simulink model "model"  (R2014a)
(part 3 of 3)

  bus4 : powerlib/Measurements/Load Flow Bus  LConnTagsString=a  ID=bus4  Vbase=132000  Vref=1  Vangle=0  VLF=1  angleLF=0
      settings: AttributesFormatString=|
      | %<ID>
      | %<Vbase>V
      | %<VLF>pu
      | %<angleLF>deg.
      | %<Name>
  bus40 : powerlib/Measurements/Load Flow Bus  LConnTagsString=a  ID=bus40  Vbase=132000  Vref=1  Vangle=0  VLF=1  angleLF=0
      settings: AttributesFormatString=|
      | %<ID>
      | %<Vbase>V
      | %<VLF>pu
      | %<angleLF>deg.
      | %<Name>
  bus41 : powerlib/Measurements/Load Flow Bus  LConnTagsString=a  ID=bus41  Vbase=132000  Vref=1  Vangle=0  VLF=1  angleLF=0
      settings: AttributesFormatString=|
      | %<ID>
      | %<Vbase>V
      | %<VLF>pu
      | %<angleLF>deg.
      | %<Name>
  bus42 : powerlib/Measurements/Load Flow Bus  LConnTagsString=a  ID=bus42  Vbase=132000  Vref=1  Vangle=0  VLF=1  angleLF=0
      settings: AttributesFormatString=|
      | %<ID>
      | %<Vbase>V
      | %<VLF>pu
      | %<angleLF>deg.
      | %<Name>
  bus43 : powerlib/Measurements/Load Flow Bus  LConnTagsString=a  ID=bus43  Vbase=132000  Vref=1  Vangle=0  VLF=1  angleLF=0
      settings: AttributesFormatString=|
      | %<ID>
      | %<Vbase>V
      | %<VLF>pu
      | %<angleLF>deg.
      | %<Name>
  bus44 : powerlib/Measurements/Load Flow Bus  LConnTagsString=a  ID=bus44  Vbase=132000  Vref=1  Vangle=0  VLF=1  angleLF=0
      settings: AttributesFormatString=|
      | %<ID>
      | %<Vbase>V
      | %<VLF>pu
      | %<angleLF>deg.
      | %<Name>
  bus45 : powerlib/Measurements/Load Flow Bus  LConnTagsString=a  ID=bus45  Vbase=132000  Vref=1  Vangle=0  VLF=1  angleLF=0
      settings: AttributesFormatString=|
      | %<ID>
      | %<Vbase>V
      | %<VLF>pu
      | %<angleLF>deg.
      | %<Name>
  bus46 : powerlib/Measurements/Load Flow Bus  LConnTagsString=a  ID=bus46  Vbase=132000  Vref=1  Vangle=0  VLF=1  angleLF=0
      settings: AttributesFormatString=|
      | %<ID>
      | %<Vbase>V
      | %<VLF>pu
      | %<angleLF>deg.
      | %<Name>
  bus47 : powerlib/Measurements/Load Flow Bus  LConnTagsString=a  ID=bus47  Vbase=132000  Vref=1  Vangle=0  VLF=1  angleLF=0
      settings: AttributesFormatString=|
      | %<ID>
      | %<Vbase>V
      | %<VLF>pu
      | %<angleLF>deg.
      | %<Name>
  bus48 : powerlib/Measurements/Load Flow Bus  LConnTagsString=a  ID=bus48  Vbase=132000  Vref=1  Vangle=0  VLF=1  angleLF=0
      settings: AttributesFormatString=|
      | %<ID>
      | %<Vbase>V
      | %<VLF>pu
      | %<angleLF>deg.
      | %<Name>
  bus49 : powerlib/Measurements/Load Flow Bus  LConnTagsString=a  ID=bus49  Vbase=132000  Vref=1  Vangle=0  VLF=1  angleLF=0
      settings: AttributesFormatString=|
      | %<ID>
      | %<Vbase>V
      | %<VLF>pu
      | %<angleLF>deg.
      | %<Name>
  bus5 : powerlib/Measurements/Load Flow Bus  LConnTagsString=a  ID=bus5  Vbase=132000  Vref=1  Vangle=0  VLF=1  angleLF=0
      settings: AttributesFormatString=|
      | %<ID>
      | %<Vbase>V
      | %<VLF>pu
      | %<angleLF>deg.
      | %<Name>
  bus50 : powerlib/Measurements/Load Flow Bus  LConnTagsString=a  ID=bus50  Vbase=132000  Vref=1  Vangle=0  VLF=1  angleLF=0
      settings: AttributesFormatString=|
      | %<ID>
      | %<Vbase>V
      | %<VLF>pu
      | %<angleLF>deg.
      | %<Name>
  bus51 : powerlib/Measurements/Load Flow Bus  LConnTagsString=a  ID=bus51  Vbase=132000  Vref=1  Vangle=0  VLF=1  angleLF=0
      settings: AttributesFormatString=|
      | %<ID>
      | %<Vbase>V
      | %<VLF>pu
      | %<angleLF>deg.
      | %<Name>
  bus52 : powerlib/Measurements/Load Flow Bus  LConnTagsString=a  ID=bus52  Vbase=132000  Vref=1  Vangle=0  VLF=1  angleLF=0
      settings: AttributesFormatString=|
      | %<ID>
      | %<Vbase>V
      | %<VLF>pu
      | %<angleLF>deg.
      | %<Name>
  bus53 : powerlib/Measurements/Load Flow Bus  LConnTagsString=a  ID=bus53  Vbase=132000  Vref=1  Vangle=0  VLF=1  angleLF=0
      settings: AttributesFormatString=|
      | %<ID>
      | %<Vbase>V
      | %<VLF>pu
      | %<angleLF>deg.
      | %<Name>
  bus54 : powerlib/Measurements/Load Flow Bus  LConnTagsString=a  ID=bus54  Vbase=132000  Vref=1  Vangle=0  VLF=1  angleLF=0
      settings: AttributesFormatString=|
      | %<ID>
      | %<Vbase>V
      | %<VLF>pu
      | %<angleLF>deg.
      | %<Name>
  bus55 : powerlib/Measurements/Load Flow Bus  LConnTagsString=a  ID=bus55  Vbase=132000  Vref=1  Vangle=0  VLF=1  angleLF=0
      settings: AttributesFormatString=|
      | %<ID>
      | %<Vbase>V
      | %<VLF>pu
      | %<angleLF>deg.
      | %<Name>
  bus56 : powerlib/Measurements/Load Flow Bus  LConnTagsString=a  ID=bus56  Vbase=132000  Vref=1  Vangle=0  VLF=1  angleLF=0
      settings: AttributesFormatString=|
      | %<ID>
      | %<Vbase>V
      | %<VLF>pu
      | %<angleLF>deg.
      | %<Name>
  bus57 : powerlib/Measurements/Load Flow Bus  LConnTagsString=a  ID=bus57  Vbase=132000  Vref=1  Vangle=0  VLF=1  angleLF=0
      settings: AttributesFormatString=|
      | %<ID>
      | %<Vbase>V
      | %<VLF>pu
      | %<angleLF>deg.
      | %<Name>
  bus58 : powerlib/Measurements/Load Flow Bus  LConnTagsString=a  ID=bus58  Vbase=132000  Vref=1  Vangle=0  VLF=1  angleLF=0
      settings: AttributesFormatString=|
      | %<ID>
      | %<Vbase>V
      | %<VLF>pu
      | %<angleLF>deg.
      | %<Name>
  bus59 : powerlib/Measurements/Load Flow Bus  LConnTagsString=a  ID=bus59  Vbase=132000  Vref=1  Vangle=0  VLF=1  angleLF=0
      settings: AttributesFormatString=|
      | %<ID>
      | %<Vbase>V
      | %<VLF>pu
      | %<angleLF>deg.
      | %<Name>
  bus6 : powerlib/Measurements/Load Flow Bus  LConnTagsString=a  ID=bus6  Vbase=132000  Vref=1  Vangle=0  VLF=1  angleLF=0
      settings: AttributesFormatString=|
      | %<ID>
      | %<Vbase>V
      | %<VLF>pu
      | %<angleLF>deg.
      | %<Name>
  bus60 : powerlib/Measurements/Load Flow Bus  LConnTagsString=a  ID=bus60  Vbase=132000  Vref=1  Vangle=0  VLF=1  angleLF=0
      settings: AttributesFormatString=|
      | %<ID>
      | %<Vbase>V
      | %<VLF>pu
      | %<angleLF>deg.
      | %<Name>
  bus61 : powerlib/Measurements/Load Flow Bus  LConnTagsString=a  ID=bus61  Vbase=132000  Vref=1  Vangle=0  VLF=1  angleLF=0
      settings: AttributesFormatString=|
      | %<ID>
      | %<Vbase>V
      | %<VLF>pu
      | %<angleLF>deg.
      | %<Name>
  bus62 : powerlib/Measurements/Load Flow Bus  LConnTagsString=a  ID=bus62  Vbase=132000  Vref=1  Vangle=0  VLF=1  angleLF=0
      settings: AttributesFormatString=|
      | %<ID>
      | %<Vbase>V
      | %<VLF>pu
      | %<angleLF>deg.
      | %<Name>
  bus63 : powerlib/Measurements/Load Flow Bus  LConnTagsString=a  ID=bus63  Vbase=132000  Vref=1  Vangle=0  VLF=1  angleLF=0
      settings: AttributesFormatString=|
      | %<ID>
      | %<Vbase>V
      | %<VLF>pu
      | %<angleLF>deg.
      | %<Name>
  bus64 : powerlib/Measurements/Load Flow Bus  LConnTagsString=a  ID=bus64  Vbase=132000  Vref=1  Vangle=0  VLF=1  angleLF=0
      settings: AttributesFormatString=|
      | %<ID>
      | %<Vbase>V
      | %<VLF>pu
      | %<angleLF>deg.
      | %<Name>
  bus65 : powerlib/Measurements/Load Flow Bus  LConnTagsString=a  ID=bus65  Vbase=132000  Vref=1  Vangle=0  VLF=1  angleLF=0
      settings: AttributesFormatString=|
      | %<ID>
      | %<Vbase>V
      | %<VLF>pu
      | %<angleLF>deg.
      | %<Name>
  bus66 : powerlib/Measurements/Load Flow Bus  LConnTagsString=a  ID=bus66  Vbase=132000  Vref=1  Vangle=0  VLF=1  angleLF=0
      settings: AttributesFormatString=|
      | %<ID>
      | %<Vbase>V
      | %<VLF>pu
      | %<angleLF>deg.
      | %<Name>
  bus67 : powerlib/Measurements/Load Flow Bus  LConnTagsString=a  ID=bus67  Vbase=132000  Vref=1  Vangle=0  VLF=1  angleLF=0
      settings: AttributesFormatString=|
      | %<ID>
      | %<Vbase>V
      | %<VLF>pu
      | %<angleLF>deg.
      | %<Name>
  bus68 : powerlib/Measurements/Load Flow Bus  LConnTagsString=a  ID=bus68  Vbase=132000  Vref=1  Vangle=0  VLF=1  angleLF=0
      settings: AttributesFormatString=|
      | %<ID>
      | %<Vbase>V
      | %<VLF>pu
      | %<angleLF>deg.
      | %<Name>
  bus69 : powerlib/Measurements/Load Flow Bus  LConnTagsString=a  ID=bus69  Vbase=132000  Vref=1  Vangle=0  VLF=1  angleLF=0
      settings: AttributesFormatString=|
      | %<ID>
      | %<Vbase>V
      | %<VLF>pu
      | %<angleLF>deg.
      | %<Name>
  bus7 : powerlib/Measurements/Load Flow Bus  LConnTagsString=a  ID=bus7  Vbase=132000  Vref=1  Vangle=0  VLF=1  angleLF=0
      settings: AttributesFormatString=|
      | %<ID>
      | %<Vbase>V
      | %<VLF>pu
      | %<angleLF>deg.
      | %<Name>
  bus70 : powerlib/Measurements/Load Flow Bus  LConnTagsString=a  ID=bus70  Vbase=132000  Vref=1  Vangle=0  VLF=1  angleLF=0
      settings: AttributesFormatString=|
      | %<ID>
      | %<Vbase>V
      | %<VLF>pu
      | %<angleLF>deg.
      | %<Name>
  bus71 : powerlib/Measurements/Load Flow Bus  LConnTagsString=a  ID=bus71  Vbase=132000  Vref=1  Vangle=0  VLF=1  angleLF=0
      settings: AttributesFormatString=|
      | %<ID>
      | %<Vbase>V
      | %<VLF>pu
      | %<angleLF>deg.
      | %<Name>
  bus72 : powerlib/Measurements/Load Flow Bus  LConnTagsString=a  ID=bus72  Vbase=132000  Vref=1  Vangle=0  VLF=1  angleLF=0
      settings: AttributesFormatString=|
      | %<ID>
      | %<Vbase>V
      | %<VLF>pu
      | %<angleLF>deg.
      | %<Name>
  bus73 : powerlib/Measurements/Load Flow Bus  LConnTagsString=a  ID=bus73  Vbase=132000  Vref=1  Vangle=0  VLF=1  angleLF=0
      settings: AttributesFormatString=|
      | %<ID>
      | %<Vbase>V
      | %<VLF>pu
      | %<angleLF>deg.
      | %<Name>
  bus74 : powerlib/Measurements/Load Flow Bus  LConnTagsString=a  ID=bus74  Vbase=132000  Vref=1  Vangle=0  VLF=1  angleLF=0
      settings: AttributesFormatString=|
      | %<ID>
      | %<Vbase>V
      | %<VLF>pu
      | %<angleLF>deg.
      | %<Name>
  bus75 : powerlib/Measurements/Load Flow Bus  LConnTagsString=a  ID=bus75  Vbase=132000  Vref=1  Vangle=0  VLF=1  angleLF=0
      settings: AttributesFormatString=|
      | %<ID>
      | %<Vbase>V
      | %<VLF>pu
      | %<angleLF>deg.
      | %<Name>
  bus76 : powerlib/Measurements/Load Flow Bus  LConnTagsString=a  ID=bus76  Vbase=132000  Vref=1  Vangle=0  VLF=1  angleLF=0
      settings: AttributesFormatString=|
      | %<ID>
      | %<Vbase>V
      | %<VLF>pu
      | %<angleLF>deg.
      | %<Name>
  bus77 : powerlib/Measurements/Load Flow Bus  LConnTagsString=a  ID=bus77  Vbase=132000  Vref=1  Vangle=0  VLF=1  angleLF=0
      settings: AttributesFormatString=|
      | %<ID>
      | %<Vbase>V
      | %<VLF>pu
      | %<angleLF>deg.
      | %<Name>
  bus78 : powerlib/Measurements/Load Flow Bus  LConnTagsString=a  ID=bus78  Vbase=132000  Vref=1  Vangle=0  VLF=1  angleLF=0
      settings: AttributesFormatString=|
      | %<ID>
      | %<Vbase>V
      | %<VLF>pu
      | %<angleLF>deg.
      | %<Name>
  bus79 : powerlib/Measurements/Load Flow Bus  LConnTagsString=a  ID=bus79  Vbase=132000  Vref=1  Vangle=0  VLF=1  angleLF=0
      settings: AttributesFormatString=|
      | %<ID>
      | %<Vbase>V
      | %<VLF>pu
      | %<angleLF>deg.
      | %<Name>
  bus8 : powerlib/Measurements/Load Flow Bus  LConnTagsString=a  ID=bus8  Vbase=132000  Vref=1  Vangle=0  VLF=1  angleLF=0
      settings: AttributesFormatString=|
      | %<ID>
      | %<Vbase>V
      | %<VLF>pu
      | %<angleLF>deg.
      | %<Name>
  bus80 : powerlib/Measurements/Load Flow Bus  LConnTagsString=a  ID=bus80  Vbase=132000  Vref=1  Vangle=0  VLF=1  angleLF=0
      settings: AttributesFormatString=|
      | %<ID>
      | %<Vbase>V
      | %<VLF>pu
      | %<angleLF>deg.
      | %<Name>
  bus81 : powerlib/Measurements/Load Flow Bus  LConnTagsString=a  ID=bus81  Vbase=132000  Vref=1  Vangle=0  VLF=1  angleLF=0
      settings: AttributesFormatString=|
      | %<ID>
      | %<Vbase>V
      | %<VLF>pu
      | %<angleLF>deg.
      | %<Name>
  bus82 : powerlib/Measurements/Load Flow Bus  LConnTagsString=a  ID=bus82  Vbase=132000  Vref=1  Vangle=0  VLF=1  angleLF=0
      settings: AttributesFormatString=|
      | %<ID>
      | %<Vbase>V
      | %<VLF>pu
      | %<angleLF>deg.
      | %<Name>
  bus83 : powerlib/Measurements/Load Flow Bus  LConnTagsString=a  ID=bus83  Vbase=132000  Vref=1  Vangle=0  VLF=1  angleLF=0
      settings: AttributesFormatString=|
      | %<ID>
      | %<Vbase>V
      | %<VLF>pu
      | %<angleLF>deg.
      | %<Name>
  bus84 : powerlib/Measurements/Load Flow Bus  LConnTagsString=a  ID=bus84  Vbase=132000  Vref=1  Vangle=0  VLF=1  angleLF=0
      settings: AttributesFormatString=|
      | %<ID>
      | %<Vbase>V
      | %<VLF>pu
      | %<angleLF>deg.
      | %<Name>
  bus85 : powerlib/Measurements/Load Flow Bus  LConnTagsString=a  ID=bus85  Vbase=132000  Vref=1  Vangle=0  VLF=1  angleLF=0
      settings: AttributesFormatString=|
      | %<ID>
      | %<Vbase>V
      | %<VLF>pu
      | %<angleLF>deg.
      | %<Name>
  bus86 : powerlib/Measurements/Load Flow Bus  LConnTagsString=a  ID=bus86  Vbase=132000  Vref=1  Vangle=0  VLF=1  angleLF=0
      settings: AttributesFormatString=|
      | %<ID>
      | %<Vbase>V
      | %<VLF>pu
      | %<angleLF>deg.
      | %<Name>
  bus87 : powerlib/Measurements/Load Flow Bus  LConnTagsString=a  ID=bus87  Vbase=132000  Vref=1  Vangle=0  VLF=1  angleLF=0
      settings: AttributesFormatString=|
      | %<ID>
      | %<Vbase>V
      | %<VLF>pu
      | %<angleLF>deg.
      | %<Name>
  bus88 : powerlib/Measurements/Load Flow Bus  LConnTagsString=a  ID=bus88  Vbase=132000  Vref=1  Vangle=0  VLF=1  angleLF=0
      settings: AttributesFormatString=|
      | %<ID>
      | %<Vbase>V
      | %<VLF>pu
      | %<angleLF>deg.
      | %<Name>
  bus89 : powerlib/Measurements/Load Flow Bus  LConnTagsString=a  ID=bus89  Vbase=132000  Vref=1  Vangle=0  VLF=1  angleLF=0
      settings: AttributesFormatString=|
      | %<ID>
      | %<Vbase>V
      | %<VLF>pu
      | %<angleLF>deg.
      | %<Name>
  bus9 : powerlib/Measurements/Load Flow Bus  LConnTagsString=a  ID=bus9  Vbase=132000  Vref=1  Vangle=0  VLF=1  angleLF=0
      settings: AttributesFormatString=|
      | %<ID>
      | %<Vbase>V
      | %<VLF>pu
      | %<angleLF>deg.
      | %<Name>
  bus90 : powerlib/Measurements/Load Flow Bus  LConnTagsString=a  ID=bus90  Vbase=132000  Vref=1  Vangle=0  VLF=1  angleLF=0
      settings: AttributesFormatString=|
      | %<ID>
      | %<Vbase>V
      | %<VLF>pu
      | %<angleLF>deg.
      | %<Name>
  bus91 : powerlib/Measurements/Load Flow Bus  LConnTagsString=a  ID=bus91  Vbase=132000  Vref=1  Vangle=0  VLF=1  angleLF=0
      settings: AttributesFormatString=|
      | %<ID>
      | %<Vbase>V
      | %<VLF>pu
      | %<angleLF>deg.
      | %<Name>
  bus92 : powerlib/Measurements/Load Flow Bus  LConnTagsString=a  ID=bus92  Vbase=132000  Vref=1  Vangle=0  VLF=1  angleLF=0
      settings: AttributesFormatString=|
      | %<ID>
      | %<Vbase>V
      | %<VLF>pu
      | %<angleLF>deg.
      | %<Name>
  bus93 : powerlib/Measurements/Load Flow Bus  LConnTagsString=a  ID=bus93  Vbase=132000  Vref=1  Vangle=0  VLF=1  angleLF=0
      settings: AttributesFormatString=|
      | %<ID>
      | %<Vbase>V
      | %<VLF>pu
      | %<angleLF>deg.
      | %<Name>
  bus94 : powerlib/Measurements/Load Flow Bus  LConnTagsString=a  ID=bus94  Vbase=132000  Vref=1  Vangle=0  VLF=1  angleLF=0
      settings: AttributesFormatString=|
      | %<ID>
      | %<Vbase>V
      | %<VLF>pu
      | %<angleLF>deg.
      | %<Name>
  bus95 : powerlib/Measurements/Load Flow Bus  LConnTagsString=a  ID=bus95  Vbase=132000  Vref=1  Vangle=0  VLF=1  angleLF=0
      settings: AttributesFormatString=|
      | %<ID>
      | %<Vbase>V
      | %<VLF>pu
      | %<angleLF>deg.
      | %<Name>
  bus96 : powerlib/Measurements/Load Flow Bus  LConnTagsString=a  ID=bus96  Vbase=132000  Vref=1  Vangle=0  VLF=1  angleLF=0
      settings: AttributesFormatString=|
      | %<ID>
      | %<Vbase>V
      | %<VLF>pu
      | %<angleLF>deg.
      | %<Name>
  bus97 : powerlib/Measurements/Load Flow Bus  LConnTagsString=a  ID=bus97  Vbase=132000  Vref=1  Vangle=0  VLF=1  angleLF=0
      settings: AttributesFormatString=|
      | %<ID>
      | %<Vbase>V
      | %<VLF>pu
      | %<angleLF>deg.
      | %<Name>
  bus98 : powerlib/Measurements/Load Flow Bus  LConnTagsString=a  ID=bus98  Vbase=132000  Vref=1  Vangle=0  VLF=1  angleLF=0
      settings: AttributesFormatString=|
      | %<ID>
      | %<Vbase>V
      | %<VLF>pu
      | %<angleLF>deg.
      | %<Name>
  bus99 : powerlib/Measurements/Load Flow Bus  LConnTagsString=a  ID=bus99  Vbase=132000  Vref=1  Vangle=0  VLF=1  angleLF=0
      settings: AttributesFormatString=|
      | %<ID>
      | %<Vbase>V
      | %<VLF>pu
      | %<angleLF>deg.
      | %<Name>
  powergui : powerlib/powergui  Priority=1  SimulationMode=Continuous  SolverType=Tustin  SampleTime=50e-6  frequency=60  SPID=off  DisableSnubberDevices=off  DisableRonSwitches=off  DisableVfSwitches=off  SwTol=0  Interpol=off  DisplayEquations=off  Ts=0  methode=off  frequencyindice=60  Pbase=100e6  ErrMax=1e-4  Iterations=50  UnitsV=kV  UnitsW=MW  FunctionMessages=off  echomessages=off  HookPort=off  EnableUseOfTLC=off  x0status=blocks  RestoreLinks=warning  ResistiveCurrentMeasurement=off  Frange=[0:2:500]  Ylog=off  Xlog=on  ShowGrid=off  save=off  variable=ZData  structure=0  ZoomFFT=off  StartTime=0.0  cycles=1  DisplayStyle=1  fundamental=60  FreqAxis=off  MaxFrequency=1000  frequencyindicesteady=1  RmsSteady=1  display=off
  connections:
  T_413160960__/LConn1 -- _CN_413160960_132000_CN_413160965_132000/LConn1
  T_413160960__/LConn2 -- _CN_413160960_132000_CN_413160965_132000/LConn2
  _CN_413160960_132000_CN_413160965_132000/LConn3 -- T_413160960__/LConn3 -- bus1/LConn1
  T_413160965__/LConn1 -- _CN_413160960_132000_CN_413160965_132000/RConn1
  T_413160965__/LConn2 -- _CN_413160960_132000_CN_413160965_132000/RConn2
  _CN_413160960_132000_CN_413160965_132000/RConn3 -- T_413160965__/LConn3 -- bus2/LConn1
  T_124680196__/LConn1 -- Puerto_Madryn___Parque_eólico_Loma_Blanca_CN_124680196_132000_CN_429400926_132000/LConn1
  T_124680196__/LConn2 -- Puerto_Madryn___Parque_eólico_Loma_Blanca_CN_124680196_132000_CN_429400926_132000/LConn2
  Puerto_Madryn___Parque_eólico_Loma_Blanca_CN_124680196_132000_CN_429400926_132000/LConn3 -- T_124680196__/LConn3 -- bus3/LConn1
  T_429400926_132000_Estación_Parque_eólico_Loma_Blanca/LConn1 -- Puerto_Madryn___Parque_eólico_Loma_Blanca_CN_124680196_132000_CN_429400926_132000/RConn1
  T_429400926_132000_Estación_Parque_eólico_Loma_Blanca/LConn2 -- Puerto_Madryn___Parque_eólico_Loma_Blanca_CN_124680196_132000_CN_429400926_132000/RConn2
  Puerto_Madryn___Parque_eólico_Loma_Blanca_CN_124680196_132000_CN_429400926_132000/RConn3 -- T_429400926_132000_Estación_Parque_eólico_Loma_Blanca/LConn3 -- bus4/LConn1
  T_313124869__/LConn1 -- _CN_313124869_132000_CN_323007043_132000/LConn1
  T_313124869__/LConn2 -- _CN_313124869_132000_CN_323007043_132000/LConn2
  _CN_313124869_132000_CN_323007043_132000/LConn3 -- T_313124869__/LConn3 -- bus5/LConn1
  _CN_313124869_132000_CN_323007043_132000/RConn1 -- T_323007043__/LConn1 -- _CN_22984932_132000_CN_323007043_132000/LConn1
  _CN_313124869_132000_CN_323007043_132000/RConn2 -- T_323007043__/LConn2 -- _CN_22984932_132000_CN_323007043_132000/LConn2
  _CN_313124869_132000_CN_323007043_132000/RConn3 -- T_323007043__/LConn3 -- _CN_22984932_132000_CN_323007043_132000/LConn3 -- bus6/LConn1
  T_193433094__Estación_transformadora_Santa_Cruz_Norte/LConn1 -- _CN_193433094_132000_CN_299759041_132000/LConn1
  T_193433094__Estación_transformadora_Santa_Cruz_Norte/LConn2 -- _CN_193433094_132000_CN_299759041_132000/LConn2
  _CN_193433094_132000_CN_299759041_132000/LConn3 -- T_193433094__Estación_transformadora_Santa_Cruz_Norte/LConn3 -- bus7/LConn1
  T_299759041__Subestación_transformadora_San_José/LConn1 -- _CN_193433094_132000_CN_299759041_132000/RConn1
  T_299759041__Subestación_transformadora_San_José/LConn2 -- _CN_193433094_132000_CN_299759041_132000/RConn2
  _CN_193433094_132000_CN_299759041_132000/RConn3 -- T_299759041__Subestación_transformadora_San_José/LConn3 -- bus8/LConn1
  T_413160968__/LConn1 -- _CN_413160968_132000_CN_400351708_132000/LConn1
  T_413160968__/LConn2 -- _CN_413160968_132000_CN_400351708_132000/LConn2
  _CN_413160968_132000_CN_400351708_132000/LConn3 -- T_413160968__/LConn3 -- bus9/LConn1
  _CN_413160968_132000_CN_400351708_132000/RConn1 -- T_400351708__Estación_transformadora_Pergamino/LConn1 -- _CN_392660851_132000_CN_400351708_132000/LConn1
  _CN_413160968_132000_CN_400351708_132000/RConn2 -- T_400351708__Estación_transformadora_Pergamino/LConn2 -- _CN_392660851_132000_CN_400351708_132000/LConn2
  _CN_413160968_132000_CN_400351708_132000/RConn3 -- T_400351708__Estación_transformadora_Pergamino/LConn3 -- _CN_392660851_132000_CN_400351708_132000/LConn3 -- bus10/LConn1
  T_413160970__/LConn1 -- _CN_413160970_132000_CN_215284916_132000/LConn1
  T_413160970__/LConn2 -- _CN_413160970_132000_CN_215284916_132000/LConn2
  _CN_413160970_132000_CN_215284916_132000/LConn3 -- T_413160970__/LConn3 -- bus11/LConn1
  _CN_413160970_132000_CN_215284916_132000/RConn1 -- T_215284916_500000_Estación_Transformadora_Campana/LConn1 -- _CN_413160978_132000_CN_215284916_132000/LConn1
  _CN_413160970_132000_CN_215284916_132000/RConn2 -- T_215284916_500000_Estación_Transformadora_Campana/LConn2 -- _CN_413160978_132000_CN_215284916_132000/LConn2
  _CN_413160970_132000_CN_215284916_132000/RConn3 -- T_215284916_500000_Estación_Transformadora_Campana/LConn3 -- _CN_413160978_132000_CN_215284916_132000/LConn3 -- bus12/LConn1
  _CN_321753613_132000_CN_274188832_132000/LConn1 -- T_321753613__/LConn1 -- _CN_321753613_132000_CN_208412024_132000/LConn1
  _CN_321753613_132000_CN_274188832_132000/LConn2 -- T_321753613__/LConn2 -- _CN_321753613_132000_CN_208412024_132000/LConn2
  _CN_321753613_132000_CN_274188832_132000/LConn3 -- T_321753613__/LConn3 -- _CN_321753613_132000_CN_208412024_132000/LConn3 -- bus13/LConn1
  _CN_321753613_132000_CN_274188832_132000/RConn1 -- T_274188832__/LConn1 -- _CN_263644686_132000_CN_274188832_132000/LConn1
  _CN_321753613_132000_CN_274188832_132000/RConn2 -- T_274188832__/LConn2 -- _CN_263644686_132000_CN_274188832_132000/LConn2
  _CN_321753613_132000_CN_274188832_132000/RConn3 -- T_274188832__/LConn3 -- _CN_263644686_132000_CN_274188832_132000/LConn3 -- bus14/LConn1
  _CN_321753613_132000_CN_208412024_132000/RConn1 -- T_208412024__Eléctrica/LConn1 -- _CN_309033575_132000_CN_208412024_132000/LConn1 -- _CN_248861779_132000_CN_208412024_132000/LConn1
  _CN_321753613_132000_CN_208412024_132000/RConn2 -- T_208412024__Eléctrica/LConn2 -- _CN_309033575_132000_CN_208412024_132000/LConn2 -- _CN_248861779_132000_CN_208412024_132000/LConn2
  _CN_321753613_132000_CN_208412024_132000/RConn3 -- T_208412024__Eléctrica/LConn3 -- _CN_309033575_132000_CN_208412024_132000/LConn3 -- bus15/LConn1 -- _CN_248861779_132000_CN_208412024_132000/LConn3
  _CN_263644686_132000_CN_254366935_132000/LConn1 -- T_263644686__/LConn1 -- _CN_263644686_132000_CN_274188832_132000/RConn1
  _CN_263644686_132000_CN_254366935_132000/LConn2 -- T_263644686__/LConn2 -- _CN_263644686_132000_CN_274188832_132000/RConn2
  _CN_263644686_132000_CN_254366935_132000/LConn3 -- T_263644686__/LConn3 -- _CN_263644686_132000_CN_274188832_132000/RConn3 -- bus16/LConn1
  T_254366935__/LConn1 -- _CN_263644686_132000_CN_254366935_132000/RConn1
  T_254366935__/LConn2 -- _CN_263644686_132000_CN_254366935_132000/RConn2
  _CN_263644686_132000_CN_254366935_132000/RConn3 -- T_254366935__/LConn3 -- bus17/LConn1
  T_348404653__/LConn1 -- _CN_348404653_132000_CN_348413858_132000/LConn1
  T_348404653__/LConn2 -- _CN_348404653_132000_CN_348413858_132000/LConn2
  _CN_348404653_132000_CN_348413858_132000/LConn3 -- T_348404653__/LConn3 -- bus18/LConn1
  _CN_348404653_132000_CN_348413858_132000/RConn1 -- T_348413858__/LConn1 -- _CN_255783500_132000_CN_348413858_132000/LConn1 -- _CN_348413858_132000_CN_154839518_132000/LConn1
  _CN_348404653_132000_CN_348413858_132000/RConn2 -- T_348413858__/LConn2 -- _CN_255783500_132000_CN_348413858_132000/LConn2 -- _CN_348413858_132000_CN_154839518_132000/LConn2
  _CN_348404653_132000_CN_348413858_132000/RConn3 -- T_348413858__/LConn3 -- _CN_255783500_132000_CN_348413858_132000/LConn3 -- _CN_348413858_132000_CN_154839518_132000/LConn3 -- bus19/LConn1
  _CN_413160978_132000_CN_413160933_132000/LConn1 -- T_413160978__/LConn1 -- _CN_413160978_132000_CN_215284916_132000/RConn1
  _CN_413160978_132000_CN_413160933_132000/LConn2 -- T_413160978__/LConn2 -- _CN_413160978_132000_CN_215284916_132000/RConn2
  _CN_413160978_132000_CN_413160933_132000/LConn3 -- T_413160978__/LConn3 -- _CN_413160978_132000_CN_215284916_132000/RConn3 -- bus20/LConn1
  T_413160933__/LConn1 -- _CN_413160978_132000_CN_413160933_132000/RConn1
  T_413160933__/LConn2 -- _CN_413160978_132000_CN_413160933_132000/RConn2
  _CN_413160978_132000_CN_413160933_132000/RConn3 -- T_413160933__/LConn3 -- bus21/LConn1
  _CN_314578968_132000_CN_267158870_132000/LConn1 -- T_314578968_132000_/LConn1 -- _CN_314578968_132000_CN_277739296_132000/LConn1 -- _CN_314578968_132000_CN_277641812_132000/LConn1 -- _CN_314578968_132000_CN_276036475_132000/LConn1
  _CN_314578968_132000_CN_267158870_132000/LConn2 -- T_314578968_132000_/LConn2 -- _CN_314578968_132000_CN_277739296_132000/LConn2 -- _CN_314578968_132000_CN_277641812_132000/LConn2 -- _CN_314578968_132000_CN_276036475_132000/LConn2
  _CN_314578968_132000_CN_267158870_132000/LConn3 -- T_314578968_132000_/LConn3 -- _CN_314578968_132000_CN_277739296_132000/LConn3 -- bus22/LConn1 -- _CN_314578968_132000_CN_277641812_132000/LConn3 -- _CN_314578968_132000_CN_276036475_132000/LConn3
  T_267158870__/LConn1 -- _CN_314578968_132000_CN_267158870_132000/RConn1
  T_267158870__/LConn2 -- _CN_314578968_132000_CN_267158870_132000/RConn2
  _CN_314578968_132000_CN_267158870_132000/RConn3 -- T_267158870__/LConn3 -- bus23/LConn1
  _CN_314578968_132000_CN_277641812_132000/RConn1 -- T_277641812__/LConn1 -- _CN_277641812_132000_CN_277641813_132000/LConn1
  _CN_314578968_132000_CN_277641812_132000/RConn2 -- T_277641812__/LConn2 -- _CN_277641812_132000_CN_277641813_132000/LConn2
  _CN_314578968_132000_CN_277641812_132000/RConn3 -- T_277641812__/LConn3 -- _CN_277641812_132000_CN_277641813_132000/LConn3 -- bus24/LConn1
  T_276036475__/LConn1 -- _CN_314578968_132000_CN_276036475_132000/RConn1
  T_276036475__/LConn2 -- _CN_314578968_132000_CN_276036475_132000/RConn2
  _CN_314578968_132000_CN_276036475_132000/RConn3 -- T_276036475__/LConn3 -- bus25/LConn1
  _CN_314578968_132000_CN_277739296_132000/RConn1 -- T_277739296_132000_/LConn1 -- _CN_277739295_132000_CN_277739296_132000/LConn1 -- _CN_277739296_132000_CN_277641813_132000/LConn1 -- _CN_277739296_132000_CN_277739298_132000/LConn1
  _CN_314578968_132000_CN_277739296_132000/RConn2 -- T_277739296_132000_/LConn2 -- _CN_277739295_132000_CN_277739296_132000/LConn2 -- _CN_277739296_132000_CN_277641813_132000/LConn2 -- _CN_277739296_132000_CN_277739298_132000/LConn2
  _CN_314578968_132000_CN_277739296_132000/RConn3 -- T_277739296_132000_/LConn3 -- _CN_277739295_132000_CN_277739296_132000/LConn3 -- _CN_277739296_132000_CN_277641813_132000/LConn3 -- _CN_277739296_132000_CN_277739298_132000/LConn3 -- bus26/LConn1
  _CN_329781274_132000_CN_188145045_132000/LConn1 -- T_329781274__/LConn1 -- _CN_329781274_132000_CN_193707888_132000/LConn1
  _CN_329781274_132000_CN_188145045_132000/LConn2 -- T_329781274__/LConn2 -- _CN_329781274_132000_CN_193707888_132000/LConn2
  _CN_329781274_132000_CN_188145045_132000/LConn3 -- T_329781274__/LConn3 -- _CN_329781274_132000_CN_193707888_132000/LConn3 -- bus27/LConn1
  T_188145045__/LConn1 -- _CN_329781274_132000_CN_188145045_132000/RConn1
  T_188145045__/LConn2 -- _CN_329781274_132000_CN_188145045_132000/RConn2
  _CN_329781274_132000_CN_188145045_132000/RConn3 -- T_188145045__/LConn3 -- bus28/LConn1
  T_193707888__/LConn1 -- _CN_329781274_132000_CN_193707888_132000/RConn1
  T_193707888__/LConn2 -- _CN_329781274_132000_CN_193707888_132000/RConn2
  _CN_329781274_132000_CN_193707888_132000/RConn3 -- T_193707888__/LConn3 -- bus29/LConn1
  _CN_194575899_132000_CN_230950275_132000/LConn1 -- T_194575899__/RConn1 -- _CN_194575899_132000_CN_213353516_132000/LConn1 -- _CN_194575899_132000_CN_214867294_132000/LConn1 -- L_194575899/LConn1
  _CN_194575899_132000_CN_230950275_132000/LConn2 -- T_194575899__/RConn2 -- _CN_194575899_132000_CN_213353516_132000/LConn2 -- _CN_194575899_132000_CN_214867294_132000/LConn2 -- L_194575899/LConn2
  _CN_194575899_132000_CN_230950275_132000/LConn3 -- T_194575899__/RConn3 -- _CN_194575899_132000_CN_213353516_132000/LConn3 -- _CN_194575899_132000_CN_214867294_132000/LConn3 -- L_194575899/LConn3 -- bus30/LConn1
  T_230950275__/LConn1 -- _CN_194575899_132000_CN_230950275_132000/RConn1
  T_230950275__/LConn2 -- _CN_194575899_132000_CN_230950275_132000/RConn2
  _CN_194575899_132000_CN_230950275_132000/RConn3 -- T_230950275__/LConn3 -- bus31/LConn1
  _CN_194575899_132000_CN_213353516_132000/RConn1 -- G_213353516_Central_Nuclear_Embalse/RConn1 -- _CN_213578175_500000_CN_213353516_132000/LConn1 -- _CN_194575899_500000_CN_213353516_132000/LConn1
  _CN_194575899_132000_CN_213353516_132000/RConn2 -- G_213353516_Central_Nuclear_Embalse/RConn2 -- _CN_213578175_500000_CN_213353516_132000/LConn2 -- _CN_194575899_500000_CN_213353516_132000/LConn2
  _CN_194575899_132000_CN_213353516_132000/RConn3 -- G_213353516_Central_Nuclear_Embalse/RConn3 -- _CN_213578175_500000_CN_213353516_132000/LConn3 -- bus32/LConn1 -- _CN_194575899_500000_CN_213353516_132000/LConn3
  T_214867294__/LConn1 -- _CN_194575899_132000_CN_214867294_132000/RConn1
  T_214867294__/LConn2 -- _CN_194575899_132000_CN_214867294_132000/RConn2
  _CN_194575899_132000_CN_214867294_132000/RConn3 -- T_214867294__/LConn3 -- bus33/LConn1
  T_251640352__Subestación_Sudeste/LConn1 -- _CN_251640352_132000_CN_251673647_132000/LConn1
  T_251640352__Subestación_Sudeste/LConn2 -- _CN_251640352_132000_CN_251673647_132000/LConn2
  _CN_251640352_132000_CN_251673647_132000/LConn3 -- T_251640352__Subestación_Sudeste/LConn3 -- bus34/LConn1
  _CN_251640352_132000_CN_251673647_132000/RConn1 -- T_251673647__Subestación_La_Plata/RConn1 -- L_251673647/LConn1
  _CN_251640352_132000_CN_251673647_132000/RConn2 -- T_251673647__Subestación_La_Plata/RConn2 -- L_251673647/LConn2
  _CN_251640352_132000_CN_251673647_132000/RConn3 -- T_251673647__Subestación_La_Plata/RConn3 -- L_251673647/LConn3 -- bus35/LConn1
  T_320719910__/LConn1 -- _CN_320719910_132000_CN_323007038_132000/LConn1
  T_320719910__/LConn2 -- _CN_320719910_132000_CN_323007038_132000/LConn2
  _CN_320719910_132000_CN_323007038_132000/LConn3 -- T_320719910__/LConn3 -- bus36/LConn1
  T_323007038__/LConn1 -- _CN_320719910_132000_CN_323007038_132000/RConn1
  T_323007038__/LConn2 -- _CN_320719910_132000_CN_323007038_132000/RConn2
  _CN_320719910_132000_CN_323007038_132000/RConn3 -- T_323007038__/LConn3 -- bus37/LConn1
  T_381521453__/LConn1 -- _CN_381521453_132000_CN_323007048_132000/LConn1
  T_381521453__/LConn2 -- _CN_381521453_132000_CN_323007048_132000/LConn2
  _CN_381521453_132000_CN_323007048_132000/LConn3 -- T_381521453__/LConn3 -- bus38/LConn1
  _CN_381521453_132000_CN_323007048_132000/RConn1 -- T_323007048__/LConn1 -- _CN_413160959_132000_CN_323007048_132000/LConn1 -- _CN_290602502_132000_CN_323007048_132000/LConn1 -- _CN_323007048_132000_CN_193415212_132000/LConn1
  _CN_381521453_132000_CN_323007048_132000/RConn2 -- T_323007048__/LConn2 -- _CN_413160959_132000_CN_323007048_132000/LConn2 -- _CN_290602502_132000_CN_323007048_132000/LConn2 -- _CN_323007048_132000_CN_193415212_132000/LConn2
  _CN_381521453_132000_CN_323007048_132000/RConn3 -- T_323007048__/LConn3 -- _CN_413160959_132000_CN_323007048_132000/LConn3 -- _CN_290602502_132000_CN_323007048_132000/LConn3 -- _CN_323007048_132000_CN_193415212_132000/LConn3 -- bus39/LConn1
  _CN_199147054_132000_CN_195246048_132000/LConn1 -- T_199147054_132000_Estación_Transformadora_Malvinas/LConn1 -- _CN_199147054_132000_CN_285751980_132000/LConn1
  _CN_199147054_132000_CN_195246048_132000/LConn2 -- T_199147054_132000_Estación_Transformadora_Malvinas/LConn2 -- _CN_199147054_132000_CN_285751980_132000/LConn2
  _CN_199147054_132000_CN_195246048_132000/LConn3 -- T_199147054_132000_Estación_Transformadora_Malvinas/LConn3 -- _CN_199147054_132000_CN_285751980_132000/LConn3 -- bus40/LConn1
  T_195246048__/LConn1 -- _CN_199147054_132000_CN_195246048_132000/RConn1
  T_195246048__/LConn2 -- _CN_199147054_132000_CN_195246048_132000/RConn2
  _CN_199147054_132000_CN_195246048_132000/RConn3 -- T_195246048__/LConn3 -- bus41/LConn1
  T_285751980_132000_Estación_Transformadora_Luján/LConn1 -- _CN_199147054_132000_CN_285751980_132000/RConn1
  T_285751980_132000_Estación_Transformadora_Luján/LConn2 -- _CN_199147054_132000_CN_285751980_132000/RConn2
  _CN_199147054_132000_CN_285751980_132000/RConn3 -- T_285751980_132000_Estación_Transformadora_Luján/LConn3 -- bus42/LConn1
  _CN_323007027_132000_CN_163331032_132000/LConn1 -- T_323007027__/LConn1 -- _CN_323007027_132000_CN_321398723_132000/LConn1
  _CN_323007027_132000_CN_163331032_132000/LConn2 -- T_323007027__/LConn2 -- _CN_323007027_132000_CN_321398723_132000/LConn2
  _CN_323007027_132000_CN_163331032_132000/LConn3 -- T_323007027__/LConn3 -- _CN_323007027_132000_CN_321398723_132000/LConn3 -- bus43/LConn1
  T_163331032__/LConn1 -- _CN_323007027_132000_CN_163331032_132000/RConn1
  T_163331032__/LConn2 -- _CN_323007027_132000_CN_163331032_132000/RConn2
  _CN_323007027_132000_CN_163331032_132000/RConn3 -- T_163331032__/LConn3 -- bus44/LConn1
  _CN_323007027_132000_CN_321398723_132000/RConn1 -- T_321398723__/RConn1 -- _CN_321398723_132000_CN_321398721_132000/LConn1 -- L_321398723/LConn1
  _CN_323007027_132000_CN_321398723_132000/RConn2 -- T_321398723__/RConn2 -- _CN_321398723_132000_CN_321398721_132000/LConn2 -- L_321398723/LConn2
  _CN_323007027_132000_CN_321398723_132000/RConn3 -- T_321398723__/RConn3 -- _CN_321398723_132000_CN_321398721_132000/LConn3 -- L_321398723/LConn3 -- bus45/LConn1
  T_323007032__/LConn1 -- _CN_323007032_132000_CN_323007054_132000/LConn1
  T_323007032__/LConn2 -- _CN_323007032_132000_CN_323007054_132000/LConn2
  _CN_323007032_132000_CN_323007054_132000/LConn3 -- T_323007032__/LConn3 -- bus46/LConn1
  _CN_323007032_132000_CN_323007054_132000/RConn1 -- T_323007054__/LConn1 -- _CN_323007054_132000_CN_272051854_132000/LConn1
  _CN_323007032_132000_CN_323007054_132000/RConn2 -- T_323007054__/LConn2 -- _CN_323007054_132000_CN_272051854_132000/LConn2
  _CN_323007032_132000_CN_323007054_132000/RConn3 -- T_323007054__/LConn3 -- _CN_323007054_132000_CN_272051854_132000/LConn3 -- bus47/LConn1
  T_413160973__/LConn1 -- _CN_413160973_132000_CN_413160958_132000/LConn1
  T_413160973__/LConn2 -- _CN_413160973_132000_CN_413160958_132000/LConn2
  _CN_413160973_132000_CN_413160958_132000/LConn3 -- T_413160973__/LConn3 -- bus48/LConn1
  _CN_413160973_132000_CN_413160958_132000/RConn1 -- T_413160958__/LConn1 -- _CN_290602502_132000_CN_413160958_132000/LConn1
  _CN_413160973_132000_CN_413160958_132000/RConn2 -- T_413160958__/LConn2 -- _CN_290602502_132000_CN_413160958_132000/LConn2
  _CN_413160973_132000_CN_413160958_132000/RConn3 -- T_413160958__/LConn3 -- _CN_290602502_132000_CN_413160958_132000/LConn3 -- bus49/LConn1
  _CN_191859780_132000_CN_323007058_132000/LConn1 -- T_191859780__/RConn1 -- L_191859780/LConn1
  _CN_191859780_132000_CN_323007058_132000/LConn2 -- T_191859780__/RConn2 -- L_191859780/LConn2
  _CN_191859780_132000_CN_323007058_132000/LConn3 -- T_191859780__/RConn3 -- L_191859780/LConn3 -- bus50/LConn1
  _CN_191859780_132000_CN_323007058_132000/RConn1 -- T_323007058__/LConn1 -- _CN_272051854_132000_CN_323007058_132000/LConn1
  _CN_191859780_132000_CN_323007058_132000/RConn2 -- T_323007058__/LConn2 -- _CN_272051854_132000_CN_323007058_132000/LConn2
  _CN_191859780_132000_CN_323007058_132000/RConn3 -- T_323007058__/LConn3 -- _CN_272051854_132000_CN_323007058_132000/LConn3 -- bus51/LConn1
  _CN_58676298_132000_CN_321536940_132000/LConn1 -- T_58676298__Subestación_Edenor/RConn1 -- _CN_58676298_132000_CN_322915916_132000/LConn1 -- L_58676298/LConn1
  _CN_58676298_132000_CN_321536940_132000/LConn2 -- T_58676298__Subestación_Edenor/RConn2 -- _CN_58676298_132000_CN_322915916_132000/LConn2 -- L_58676298/LConn2
  _CN_58676298_132000_CN_321536940_132000/LConn3 -- T_58676298__Subestación_Edenor/RConn3 -- _CN_58676298_132000_CN_322915916_132000/LConn3 -- L_58676298/LConn3 -- bus52/LConn1
  T_321536940__/LConn1 -- _CN_58676298_132000_CN_321536940_132000/RConn1
  T_321536940__/LConn2 -- _CN_58676298_132000_CN_321536940_132000/RConn2
  _CN_58676298_132000_CN_321536940_132000/RConn3 -- T_321536940__/LConn3 -- bus53/LConn1
  T_322915916__/LConn1 -- _CN_58676298_132000_CN_322915916_132000/RConn1
  T_322915916__/LConn2 -- _CN_58676298_132000_CN_322915916_132000/RConn2
  _CN_58676298_132000_CN_322915916_132000/RConn3 -- T_322915916__/LConn3 -- bus54/LConn1
  _CN_255783500_132000_CN_277739294_132000/LConn1 -- T_255783500__/LConn1 -- _CN_255783500_132000_CN_314623617_132000/LConn1 -- _CN_255783500_132000_CN_183904319_132000/LConn1 -- _CN_255783500_132000_CN_348409732_132000/LConn1 -- _CN_255783500_132000_CN_348413858_132000/RConn1
  _CN_255783500_132000_CN_277739294_132000/LConn2 -- T_255783500__/LConn2 -- _CN_255783500_132000_CN_314623617_132000/LConn2 -- _CN_255783500_132000_CN_183904319_132000/LConn2 -- _CN_255783500_132000_CN_348409732_132000/LConn2 -- _CN_255783500_132000_CN_348413858_132000/RConn2
  _CN_255783500_132000_CN_277739294_132000/LConn3 -- T_255783500__/LConn3 -- _CN_255783500_132000_CN_314623617_132000/LConn3 -- _CN_255783500_132000_CN_183904319_132000/LConn3 -- _CN_255783500_132000_CN_348409732_132000/LConn3 -- _CN_255783500_132000_CN_348413858_132000/RConn3 -- bus55/LConn1
  _CN_255783500_132000_CN_277739294_132000/RConn1 -- T_277739294__/LConn1 -- _CN_277739294_132000_CN_277739297_132000/LConn1
  _CN_255783500_132000_CN_277739294_132000/RConn2 -- T_277739294__/LConn2 -- _CN_277739294_132000_CN_277739297_132000/LConn2
  _CN_255783500_132000_CN_277739294_132000/RConn3 -- T_277739294__/LConn3 -- _CN_277739294_132000_CN_277739297_132000/LConn3 -- bus56/LConn1
  T_314623617__/LConn1 -- _CN_255783500_132000_CN_314623617_132000/RConn1
  T_314623617__/LConn2 -- _CN_255783500_132000_CN_314623617_132000/RConn2
  _CN_255783500_132000_CN_314623617_132000/RConn3 -- T_314623617__/LConn3 -- bus57/LConn1
  G_183904319_Central_Termoeléctrica_Necochea/RConn1 -- _CN_255783500_132000_CN_183904319_132000/RConn1
  G_183904319_Central_Termoeléctrica_Necochea/RConn2 -- _CN_255783500_132000_CN_183904319_132000/RConn2
  _CN_255783500_132000_CN_183904319_132000/RConn3 -- G_183904319_Central_Termoeléctrica_Necochea/RConn3 -- bus58/LConn1
  T_348409732__/LConn1 -- _CN_255783500_132000_CN_348409732_132000/RConn1
  T_348409732__/LConn2 -- _CN_255783500_132000_CN_348409732_132000/RConn2
  _CN_255783500_132000_CN_348409732_132000/RConn3 -- T_348409732__/LConn3 -- bus59/LConn1
  _CN_323007054_132000_CN_272051854_132000/RConn1 -- T_272051854__/RConn1 -- _CN_272051854_132000_CN_310571477_132000/LConn1 -- L_272051854/LConn1 -- _CN_272051854_132000_CN_323007058_132000/RConn1
  _CN_323007054_132000_CN_272051854_132000/RConn2 -- T_272051854__/RConn2 -- _CN_272051854_132000_CN_310571477_132000/LConn2 -- L_272051854/LConn2 -- _CN_272051854_132000_CN_323007058_132000/RConn2
  _CN_323007054_132000_CN_272051854_132000/RConn3 -- T_272051854__/RConn3 -- _CN_272051854_132000_CN_310571477_132000/LConn3 -- L_272051854/LConn3 -- bus60/LConn1 -- _CN_272051854_132000_CN_323007058_132000/RConn3
  _CN_193412175_132000_CN_323007050_132000/LConn1 -- T_193412175_500000_Estación_transformadora_Ramallo/RConn4 -- L_193412175/LConn1
  _CN_193412175_132000_CN_323007050_132000/LConn2 -- T_193412175_500000_Estación_transformadora_Ramallo/RConn5 -- L_193412175/LConn2
  _CN_193412175_132000_CN_323007050_132000/LConn3 -- T_193412175_500000_Estación_transformadora_Ramallo/RConn6 -- L_193412175/LConn3 -- bus61/LConn1
  _CN_193412175_132000_CN_323007050_132000/RConn1 -- T_323007050__/LConn1 -- _CN_290602502_132000_CN_323007050_132000/LConn1
  _CN_193412175_132000_CN_323007050_132000/RConn2 -- T_323007050__/LConn2 -- _CN_290602502_132000_CN_323007050_132000/LConn2
  _CN_193412175_132000_CN_323007050_132000/RConn3 -- T_323007050__/LConn3 -- _CN_290602502_132000_CN_323007050_132000/LConn3 -- bus62/LConn1
  T_204494929__Estação_Conversora_de_Frequencia_de_Uruguaiana/LConn1 -- _CN_204494929_132000_CN_204494933_132000/LConn1
  T_204494929__Estação_Conversora_de_Frequencia_de_Uruguaiana/LConn2 -- _CN_204494929_132000_CN_204494933_132000/LConn2
  _CN_204494929_132000_CN_204494933_132000/LConn3 -- T_204494929__Estação_Conversora_de_Frequencia_de_Uruguaiana/LConn3 -- bus63/LConn1
  T_204494933__/LConn1 -- _CN_204494929_132000_CN_204494933_132000/RConn1
  T_204494933__/LConn2 -- _CN_204494929_132000_CN_204494933_132000/RConn2
  _CN_204494929_132000_CN_204494933_132000/RConn3 -- T_204494933__/LConn3 -- bus64/LConn1
  _CN_248861779_132000_CN_208412024_132000/RConn1 -- T_248861779__/LConn1 -- _CN_248861779_132000_CN_323105942_132000/LConn1
  _CN_248861779_132000_CN_208412024_132000/RConn2 -- T_248861779__/LConn2 -- _CN_248861779_132000_CN_323105942_132000/LConn2
  _CN_248861779_132000_CN_208412024_132000/RConn3 -- T_248861779__/LConn3 -- _CN_248861779_132000_CN_323105942_132000/LConn3 -- bus65/LConn1
  _CN_248861779_132000_CN_323105942_132000/RConn1 -- T_323105942__/LConn1 -- _CN_145419356_132000_CN_323105942_132000/LConn1
  _CN_248861779_132000_CN_323105942_132000/RConn2 -- T_323105942__/LConn2 -- _CN_145419356_132000_CN_323105942_132000/LConn2
  _CN_248861779_132000_CN_323105942_132000/RConn3 -- T_323105942__/LConn3 -- _CN_145419356_132000_CN_323105942_132000/LConn3 -- bus66/LConn1
  _CN_277641812_132000_CN_277641813_132000/RConn1 -- T_277641813__/RConn1 -- _CN_432044715_132000_CN_277641813_132000/LConn1 -- _CN_277739296_132000_CN_277641813_132000/RConn1 -- L_277641813/LConn1
  _CN_277641812_132000_CN_277641813_132000/RConn2 -- T_277641813__/RConn2 -- _CN_432044715_132000_CN_277641813_132000/LConn2 -- _CN_277739296_132000_CN_277641813_132000/RConn2 -- L_277641813/LConn2
  _CN_277641812_132000_CN_277641813_132000/RConn3 -- T_277641813__/RConn3 -- _CN_432044715_132000_CN_277641813_132000/LConn3 -- _CN_277739296_132000_CN_277641813_132000/RConn3 -- L_277641813/LConn3 -- bus67/LConn1
  _CN_145419356_132000_CN_422118006_132000/LConn1 -- T_145419356__/LConn1 -- _CN_145419356_132000_CN_130194705_132000/LConn1 -- _CN_145419356_132000_CN_323105942_132000/RConn1
  _CN_145419356_132000_CN_422118006_132000/LConn2 -- T_145419356__/LConn2 -- _CN_145419356_132000_CN_130194705_132000/LConn2 -- _CN_145419356_132000_CN_323105942_132000/RConn2
  _CN_145419356_132000_CN_422118006_132000/LConn3 -- T_145419356__/LConn3 -- _CN_145419356_132000_CN_130194705_132000/LConn3 -- _CN_145419356_132000_CN_323105942_132000/RConn3 -- bus68/LConn1
  T_422118006__/LConn1 -- _CN_145419356_132000_CN_422118006_132000/RConn1
  T_422118006__/LConn2 -- _CN_145419356_132000_CN_422118006_132000/RConn2
  _CN_145419356_132000_CN_422118006_132000/RConn3 -- T_422118006__/LConn3 -- bus69/LConn1
  _CN_145419356_132000_CN_130194705_132000/RConn1 -- T_130194705__/LConn1 -- _CN_130194705_132000_CN_154839518_132000/LConn1
  _CN_145419356_132000_CN_130194705_132000/RConn2 -- T_130194705__/LConn2 -- _CN_130194705_132000_CN_154839518_132000/LConn2
  _CN_145419356_132000_CN_130194705_132000/RConn3 -- T_130194705__/LConn3 -- _CN_130194705_132000_CN_154839518_132000/LConn3 -- bus70/LConn1
  T_284287249__Subestación_Sobral/LConn1 -- _CN_284287249_132000_CN_277938914_132000/LConn1
  T_284287249__Subestación_Sobral/LConn2 -- _CN_284287249_132000_CN_277938914_132000/LConn2
  _CN_284287249_132000_CN_277938914_132000/LConn3 -- T_284287249__Subestación_Sobral/LConn3 -- bus71/LConn1
  T_277938914__/LConn1 -- _CN_284287249_132000_CN_277938914_132000/RConn1
  T_277938914__/LConn2 -- _CN_284287249_132000_CN_277938914_132000/RConn2
  _CN_284287249_132000_CN_277938914_132000/RConn3 -- T_277938914__/LConn3 -- bus72/LConn1
  _CN_309033575_132000_CN_251093639_132000/LConn1 -- T_309033575__/LConn1 -- _CN_309033575_132000_CN_208412024_132000/RConn1
  _CN_309033575_132000_CN_251093639_132000/LConn2 -- T_309033575__/LConn2 -- _CN_309033575_132000_CN_208412024_132000/RConn2
  _CN_309033575_132000_CN_251093639_132000/LConn3 -- T_309033575__/LConn3 -- _CN_309033575_132000_CN_208412024_132000/RConn3 -- bus73/LConn1
  T_251093639_132000_Estación_Transformadora_Verónica/LConn1 -- _CN_309033575_132000_CN_251093639_132000/RConn1
  T_251093639_132000_Estación_Transformadora_Verónica/LConn2 -- _CN_309033575_132000_CN_251093639_132000/RConn2
  _CN_309033575_132000_CN_251093639_132000/RConn3 -- T_251093639_132000_Estación_Transformadora_Verónica/LConn3 -- bus74/LConn1
  _CN_299924594_132000_CN_223678069_132000/LConn1 -- T_299924594__Estación_Pico_Truncado_I/LConn1 -- _CN_299924594_132000_CN_299598854_132000/LConn1
  _CN_299924594_132000_CN_223678069_132000/LConn2 -- T_299924594__Estación_Pico_Truncado_I/LConn2 -- _CN_299924594_132000_CN_299598854_132000/LConn2
  _CN_299924594_132000_CN_223678069_132000/LConn3 -- T_299924594__Estación_Pico_Truncado_I/LConn3 -- _CN_299924594_132000_CN_299598854_132000/LConn3 -- bus75/LConn1
  T_223678069__Estación_transformadora_Puerto_Deseado/LConn1 -- _CN_299924594_132000_CN_223678069_132000/RConn1
  T_223678069__Estación_transformadora_Puerto_Deseado/LConn2 -- _CN_299924594_132000_CN_223678069_132000/RConn2
  _CN_299924594_132000_CN_223678069_132000/RConn3 -- T_223678069__Estación_transformadora_Puerto_Deseado/LConn3 -- bus76/LConn1
  _CN_299924594_132000_CN_299598854_132000/RConn1 -- T_299598854__Estación_transformadora_Las_Heras/LConn1 -- _CN_299598854_132000_CN_317981558_132000/LConn1
  _CN_299924594_132000_CN_299598854_132000/RConn2 -- T_299598854__Estación_transformadora_Las_Heras/LConn2 -- _CN_299598854_132000_CN_317981558_132000/LConn2
  _CN_299924594_132000_CN_299598854_132000/RConn3 -- T_299598854__Estación_transformadora_Las_Heras/LConn3 -- _CN_299598854_132000_CN_317981558_132000/LConn3 -- bus77/LConn1
  T_129988212__Subestación_Transformadora_Transba/LConn1 -- _CN_129988212_132000_CN_257673618_132000/LConn1
  T_129988212__Subestación_Transformadora_Transba/LConn2 -- _CN_129988212_132000_CN_257673618_132000/LConn2
  _CN_129988212_132000_CN_257673618_132000/LConn3 -- T_129988212__Subestación_Transformadora_Transba/LConn3 -- bus78/LConn1
  _CN_129988212_132000_CN_257673618_132000/RConn1 -- T_257673618__/RConn1 -- _CN_257673618_132000_CN_154839518_132000/LConn1 -- L_257673618/LConn1
  _CN_129988212_132000_CN_257673618_132000/RConn2 -- T_257673618__/RConn2 -- _CN_257673618_132000_CN_154839518_132000/LConn2 -- L_257673618/LConn2
  _CN_129988212_132000_CN_257673618_132000/RConn3 -- T_257673618__/RConn3 -- _CN_257673618_132000_CN_154839518_132000/LConn3 -- L_257673618/LConn3 -- bus79/LConn1
  T_322781304__/LConn1 -- _CN_322781304_132000_CN_208425737_132000/LConn1
  T_322781304__/LConn2 -- _CN_322781304_132000_CN_208425737_132000/LConn2
  _CN_322781304_132000_CN_208425737_132000/LConn3 -- T_322781304__/LConn3 -- bus80/LConn1
  _CN_322781304_132000_CN_208425737_132000/RConn1 -- T_208425737__Eléctrica/LConn1 -- _CN_208425737_132000_CN_22984932_132000/LConn1 -- _CN_208425737_132000_CN_431767371_132000/LConn1 -- _CN_208425737_132000_CN_241864152_132000/LConn1
  _CN_322781304_132000_CN_208425737_132000/RConn2 -- T_208425737__Eléctrica/LConn2 -- _CN_208425737_132000_CN_22984932_132000/LConn2 -- _CN_208425737_132000_CN_431767371_132000/LConn2 -- _CN_208425737_132000_CN_241864152_132000/LConn2
  _CN_322781304_132000_CN_208425737_132000/RConn3 -- T_208425737__Eléctrica/LConn3 -- _CN_208425737_132000_CN_22984932_132000/LConn3 -- _CN_208425737_132000_CN_431767371_132000/LConn3 -- _CN_208425737_132000_CN_241864152_132000/LConn3 -- bus81/LConn1
  T_210279051__Estación_Transformadora/LConn1 -- _CN_210279051_132000_CN_283604831_132000/LConn1
  T_210279051__Estación_Transformadora/LConn2 -- _CN_210279051_132000_CN_283604831_132000/LConn2
  _CN_210279051_132000_CN_283604831_132000/LConn3 -- T_210279051__Estación_Transformadora/LConn3 -- bus82/LConn1
  T_283604831__/LConn1 -- _CN_210279051_132000_CN_283604831_132000/RConn1
  T_283604831__/LConn2 -- _CN_210279051_132000_CN_283604831_132000/RConn2
  _CN_210279051_132000_CN_283604831_132000/RConn3 -- T_283604831__/LConn3 -- bus83/LConn1
  _CN_272051854_132000_CN_310571477_132000/RConn1 -- T_310571477__/LConn1 -- _CN_286336657_132000_CN_310571477_132000/LConn1
  _CN_272051854_132000_CN_310571477_132000/RConn2 -- T_310571477__/LConn2 -- _CN_286336657_132000_CN_310571477_132000/LConn2
  _CN_272051854_132000_CN_310571477_132000/RConn3 -- T_310571477__/LConn3 -- _CN_286336657_132000_CN_310571477_132000/LConn3 -- bus84/LConn1
  T_286336657__/LConn1 -- _CN_286336657_132000_CN_310571477_132000/RConn1
  T_286336657__/LConn2 -- _CN_286336657_132000_CN_310571477_132000/RConn2
  _CN_286336657_132000_CN_310571477_132000/RConn3 -- T_286336657__/LConn3 -- bus85/LConn1
  T_413160959__/LConn1 -- _CN_413160959_132000_CN_323007048_132000/RConn1
  T_413160959__/LConn2 -- _CN_413160959_132000_CN_323007048_132000/RConn2
  _CN_413160959_132000_CN_323007048_132000/RConn3 -- T_413160959__/LConn3 -- bus86/LConn1
  T_196031429__/LConn1 -- _CN_196031429_132000_CN_353728814_132000/LConn1
  T_196031429__/LConn2 -- _CN_196031429_132000_CN_353728814_132000/LConn2
  _CN_196031429_132000_CN_353728814_132000/LConn3 -- T_196031429__/LConn3 -- bus87/LConn1
  T_353728814__Estaciòn_Transformadora_San_Miguel/LConn1 -- _CN_196031429_132000_CN_353728814_132000/RConn1
  T_353728814__Estaciòn_Transformadora_San_Miguel/LConn2 -- _CN_196031429_132000_CN_353728814_132000/RConn2
  _CN_196031429_132000_CN_353728814_132000/RConn3 -- T_353728814__Estaciòn_Transformadora_San_Miguel/LConn3 -- bus88/LConn1
  _CN_290602502_132000_CN_413160958_132000/RConn1 -- T_290602502__/LConn1 -- _CN_290602502_132000_CN_323007050_132000/RConn1 -- _CN_290602502_132000_CN_323007048_132000/RConn1
  _CN_290602502_132000_CN_413160958_132000/RConn2 -- T_290602502__/LConn2 -- _CN_290602502_132000_CN_323007050_132000/RConn2 -- _CN_290602502_132000_CN_323007048_132000/RConn2
  _CN_290602502_132000_CN_413160958_132000/RConn3 -- T_290602502__/LConn3 -- _CN_290602502_132000_CN_323007050_132000/RConn3 -- bus89/LConn1 -- _CN_290602502_132000_CN_323007048_132000/RConn3
  _CN_432044715_132000_CN_431976152_132000/LConn1 -- T_432044715__/LConn1 -- _CN_432044715_132000_CN_277641813_132000/RConn1
  _CN_432044715_132000_CN_431976152_132000/LConn2 -- T_432044715__/LConn2 -- _CN_432044715_132000_CN_277641813_132000/RConn2
  _CN_432044715_132000_CN_431976152_132000/LConn3 -- T_432044715__/LConn3 -- _CN_432044715_132000_CN_277641813_132000/RConn3 -- bus90/LConn1
  T_431976152__/LConn1 -- _CN_432044715_132000_CN_431976152_132000/RConn1
  T_431976152__/LConn2 -- _CN_432044715_132000_CN_431976152_132000/RConn2
  _CN_432044715_132000_CN_431976152_132000/RConn3 -- T_431976152__/LConn3 -- bus91/LConn1
  T_306029239__/LConn1 -- _CN_306029239_132000_CN_329781271_132000/LConn1
  T_306029239__/LConn2 -- _CN_306029239_132000_CN_329781271_132000/LConn2
  _CN_306029239_132000_CN_329781271_132000/LConn3 -- T_306029239__/LConn3 -- bus92/LConn1
  T_329781271__/LConn1 -- _CN_306029239_132000_CN_329781271_132000/RConn1
  T_329781271__/LConn2 -- _CN_306029239_132000_CN_329781271_132000/RConn2
  _CN_306029239_132000_CN_329781271_132000/RConn3 -- T_329781271__/LConn3 -- bus93/LConn1
  Trelew___Rawson_CN_429251282_132000_CN_429251283_132000/LConn1 -- T_429251282_132000_Estación_Rawson/LConn1 -- Parque_eólico_Rawson___Rawson_CN_429251282_132000_CN_429251281_132000/LConn1
  Trelew___Rawson_CN_429251282_132000_CN_429251283_132000/LConn2 -- T_429251282_132000_Estación_Rawson/LConn2 -- Parque_eólico_Rawson___Rawson_CN_429251282_132000_CN_429251281_132000/LConn2
  Trelew___Rawson_CN_429251282_132000_CN_429251283_132000/LConn3 -- T_429251282_132000_Estación_Rawson/LConn3 -- Parque_eólico_Rawson___Rawson_CN_429251282_132000_CN_429251281_132000/LConn3 -- bus94/LConn1
  T_429251283_132000_Estación_Trelew/LConn1 -- Trelew___Rawson_CN_429251282_132000_CN_429251283_132000/RConn1
  T_429251283_132000_Estación_Trelew/LConn2 -- Trelew___Rawson_CN_429251282_132000_CN_429251283_132000/RConn2
  Trelew___Rawson_CN_429251282_132000_CN_429251283_132000/RConn3 -- T_429251283_132000_Estación_Trelew/LConn3 -- bus95/LConn1
  T_429251281_132000_Estación_Parque_eólico_Rawson/LConn1 -- Parque_eólico_Rawson___Rawson_CN_429251282_132000_CN_429251281_132000/RConn1
  T_429251281_132000_Estación_Parque_eólico_Rawson/LConn2 -- Parque_eólico_Rawson___Rawson_CN_429251282_132000_CN_429251281_132000/RConn2
  Parque_eólico_Rawson___Rawson_CN_429251282_132000_CN_429251281_132000/RConn3 -- T_429251281_132000_Estación_Parque_eólico_Rawson/LConn3 -- bus96/LConn1
  T_317981558__Subestación_transformadora_Los_Perales_2/LConn1 -- _CN_299598854_132000_CN_317981558_132000/RConn1
  T_317981558__Subestación_transformadora_Los_Perales_2/LConn2 -- _CN_299598854_132000_CN_317981558_132000/RConn2
  _CN_299598854_132000_CN_317981558_132000/RConn3 -- T_317981558__Subestación_transformadora_Los_Perales_2/LConn3 -- bus97/LConn1
  T_277938913__/LConn1 -- _CN_277938913_132000_CN_277938915_132000/LConn1
  T_277938913__/LConn2 -- _CN_277938913_132000_CN_277938915_132000/LConn2
  _CN_277938913_132000_CN_277938915_132000/LConn3 -- T_277938913__/LConn3 -- bus98/LConn1
  T_277938915__/LConn1 -- _CN_277938913_132000_CN_277938915_132000/RConn1
  T_277938915__/LConn2 -- _CN_277938913_132000_CN_277938915_132000/RConn2
  _CN_277938913_132000_CN_277938915_132000/RConn3 -- T_277938915__/LConn3 -- bus99/LConn1
  _CN_203363075_132000_CN_321354632_132000/LConn1 -- T_203363075__/RConn1 -- L_203363075/LConn1
  _CN_203363075_132000_CN_321354632_132000/LConn2 -- T_203363075__/RConn2 -- L_203363075/LConn2
  _CN_203363075_132000_CN_321354632_132000/LConn3 -- T_203363075__/RConn3 -- L_203363075/LConn3 -- bus100/LConn1
  T_321354632__/LConn1 -- _CN_203363075_132000_CN_321354632_132000/RConn1
  T_321354632__/LConn2 -- _CN_203363075_132000_CN_321354632_132000/RConn2
  _CN_203363075_132000_CN_321354632_132000/RConn3 -- T_321354632__/LConn3 -- bus101/LConn1
  _CN_328056071_132000_CN_363050268_132000/LConn1 -- T_328056071__/LConn1 -- _CN_328056071_132000_CN_248651545_132000/LConn1
  _CN_328056071_132000_CN_363050268_132000/LConn2 -- T_328056071__/LConn2 -- _CN_328056071_132000_CN_248651545_132000/LConn2
  _CN_328056071_132000_CN_363050268_132000/LConn3 -- T_328056071__/LConn3 -- _CN_328056071_132000_CN_248651545_132000/LConn3 -- bus102/LConn1
  _CN_328056071_132000_CN_363050268_132000/RConn1 -- T_363050268__Estacion_Transformadora_Villa_Mercedes/LConn1 -- _CN_363050268_132000_CN_211179868_132000/LConn1
  _CN_328056071_132000_CN_363050268_132000/RConn2 -- T_363050268__Estacion_Transformadora_Villa_Mercedes/LConn2 -- _CN_363050268_132000_CN_211179868_132000/LConn2
  _CN_328056071_132000_CN_363050268_132000/RConn3 -- T_363050268__Estacion_Transformadora_Villa_Mercedes/LConn3 -- _CN_363050268_132000_CN_211179868_132000/LConn3 -- bus103/LConn1
  T_248651545__/LConn1 -- _CN_328056071_132000_CN_248651545_132000/RConn1
  T_248651545__/LConn2 -- _CN_328056071_132000_CN_248651545_132000/RConn2
  _CN_328056071_132000_CN_248651545_132000/RConn3 -- T_248651545__/LConn3 -- bus104/LConn1
  _CN_208425737_132000_CN_22984932_132000/RConn1 -- T_22984932__Subestación_de_EDELAP/LConn1 -- _CN_22984932_132000_CN_323007043_132000/RConn1
  _CN_208425737_132000_CN_22984932_132000/RConn2 -- T_22984932__Subestación_de_EDELAP/LConn2 -- _CN_22984932_132000_CN_323007043_132000/RConn2
  _CN_208425737_132000_CN_22984932_132000/RConn3 -- T_22984932__Subestación_de_EDELAP/LConn3 -- _CN_22984932_132000_CN_323007043_132000/RConn3 -- bus105/LConn1
  T_431767371__/LConn1 -- _CN_208425737_132000_CN_431767371_132000/RConn1
  T_431767371__/LConn2 -- _CN_208425737_132000_CN_431767371_132000/RConn2
  _CN_208425737_132000_CN_431767371_132000/RConn3 -- T_431767371__/LConn3 -- bus106/LConn1
  T_241864152__/LConn1 -- _CN_208425737_132000_CN_241864152_132000/RConn1
  T_241864152__/LConn2 -- _CN_208425737_132000_CN_241864152_132000/RConn2
  _CN_208425737_132000_CN_241864152_132000/RConn3 -- T_241864152__/LConn3 -- bus107/LConn1
  _CN_130194705_132000_CN_154839518_132000/RConn1 -- T_154839518__TRANSBA___Subestación_Olavarría___132kV/LConn1 -- _CN_348413858_132000_CN_154839518_132000/RConn1 -- _CN_257673618_132000_CN_154839518_132000/RConn1
  _CN_130194705_132000_CN_154839518_132000/RConn2 -- T_154839518__TRANSBA___Subestación_Olavarría___132kV/LConn2 -- _CN_348413858_132000_CN_154839518_132000/RConn2 -- _CN_257673618_132000_CN_154839518_132000/RConn2
  _CN_130194705_132000_CN_154839518_132000/RConn3 -- T_154839518__TRANSBA___Subestación_Olavarría___132kV/LConn3 -- _CN_348413858_132000_CN_154839518_132000/RConn3 -- bus108/LConn1 -- _CN_257673618_132000_CN_154839518_132000/RConn3
  T_211179868__/LConn1 -- _CN_363050268_132000_CN_211179868_132000/RConn1
  T_211179868__/LConn2 -- _CN_363050268_132000_CN_211179868_132000/RConn2
  _CN_363050268_132000_CN_211179868_132000/RConn3 -- T_211179868__/LConn3 -- bus109/LConn1
  _CN_277739294_132000_CN_277739297_132000/RConn1 -- T_277739297__/LConn1 -- _CN_277739297_132000_CN_277739298_132000/LConn1
  _CN_277739294_132000_CN_277739297_132000/RConn2 -- T_277739297__/LConn2 -- _CN_277739297_132000_CN_277739298_132000/LConn2
  _CN_277739294_132000_CN_277739297_132000/RConn3 -- T_277739297__/LConn3 -- _CN_277739297_132000_CN_277739298_132000/LConn3 -- bus110/LConn1
  T_277739295_132000_/LConn1 -- _CN_277739295_132000_CN_277739296_132000/RConn1
  T_277739295_132000_/LConn2 -- _CN_277739295_132000_CN_277739296_132000/RConn2
  _CN_277739295_132000_CN_277739296_132000/RConn3 -- T_277739295_132000_/LConn3 -- bus111/LConn1
  _CN_277739296_132000_CN_277739298_132000/RConn1 -- T_277739298__/LConn1 -- _CN_277739297_132000_CN_277739298_132000/RConn1
  _CN_277739296_132000_CN_277739298_132000/RConn2 -- T_277739298__/LConn2 -- _CN_277739297_132000_CN_277739298_132000/RConn2
  _CN_277739296_132000_CN_277739298_132000/RConn3 -- T_277739298__/LConn3 -- _CN_277739297_132000_CN_277739298_132000/RConn3 -- bus112/LConn1
  _CN_179545958_132000_CN_321354631_132000/LConn1 -- T_179545958_500000_Estación_Transformadora_Ezeiza/RConn4 -- L_179545958/LConn1
  _CN_179545958_132000_CN_321354631_132000/LConn2 -- T_179545958_500000_Estación_Transformadora_Ezeiza/RConn5 -- L_179545958/LConn2
  _CN_179545958_132000_CN_321354631_132000/LConn3 -- T_179545958_500000_Estación_Transformadora_Ezeiza/RConn6 -- L_179545958/LConn3 -- bus113/LConn1
  T_321354631__/LConn1 -- _CN_179545958_132000_CN_321354631_132000/RConn1
  T_321354631__/LConn2 -- _CN_179545958_132000_CN_321354631_132000/RConn2
  _CN_179545958_132000_CN_321354631_132000/RConn3 -- T_321354631__/LConn3 -- bus114/LConn1
  T_340060050_500000_Estación_Transformadora_Centro/LConn1 -- _CN_340060050_132000_CN_97399680_132000/LConn1
  T_340060050_500000_Estación_Transformadora_Centro/LConn2 -- _CN_340060050_132000_CN_97399680_132000/LConn2
  _CN_340060050_132000_CN_97399680_132000/LConn3 -- T_340060050_500000_Estación_Transformadora_Centro/LConn3 -- bus115/LConn1
  T_97399680_500000_Estación_Transformadora_San_Isidro/LConn1 -- _CN_340060050_132000_CN_97399680_132000/RConn1
  T_97399680_500000_Estación_Transformadora_San_Isidro/LConn2 -- _CN_340060050_132000_CN_97399680_132000/RConn2
  _CN_340060050_132000_CN_97399680_132000/RConn3 -- T_97399680_500000_Estación_Transformadora_San_Isidro/LConn3 -- bus116/LConn1
  T_392660851__/LConn1 -- _CN_392660851_132000_CN_400351708_132000/RConn1
  T_392660851__/LConn2 -- _CN_392660851_132000_CN_400351708_132000/RConn2
  _CN_392660851_132000_CN_400351708_132000/RConn3 -- T_392660851__/LConn3 -- bus117/LConn1
  T_326097046__/LConn1 -- _CN_326097046_132000_CN_314176103_132000/LConn1
  T_326097046__/LConn2 -- _CN_326097046_132000_CN_314176103_132000/LConn2
  _CN_326097046_132000_CN_314176103_132000/LConn3 -- T_326097046__/LConn3 -- bus118/LConn1
  _CN_326097046_132000_CN_314176103_132000/RConn1 -- T_314176103__Estación_transformadora_Esperanza/RConn1 -- L_314176103/LConn1
  _CN_326097046_132000_CN_314176103_132000/RConn2 -- T_314176103__Estación_transformadora_Esperanza/RConn2 -- L_314176103/LConn2
  _CN_326097046_132000_CN_314176103_132000/RConn3 -- T_314176103__Estación_transformadora_Esperanza/RConn3 -- L_314176103/LConn3 -- bus119/LConn1
  T_230329765__/LConn1 -- _CN_230329765_132000_CN_322781303_132000/LConn1
  T_230329765__/LConn2 -- _CN_230329765_132000_CN_322781303_132000/LConn2
  _CN_230329765_132000_CN_322781303_132000/LConn3 -- T_230329765__/LConn3 -- bus120/LConn1
  T_322781303__/LConn1 -- _CN_230329765_132000_CN_322781303_132000/RConn1
  T_322781303__/LConn2 -- _CN_230329765_132000_CN_322781303_132000/RConn2
  _CN_230329765_132000_CN_322781303_132000/RConn3 -- T_322781303__/LConn3 -- bus121/LConn1
  _CN_323007048_132000_CN_193415212_132000/RConn1 -- G_193415212_Central_Nuclear_de_Atucha_I/RConn1 -- 2ATVL1Y2_CN_277132135_220000_CN_193415212_132000/LConn1 -- _CN_193412175_500000_CN_193415212_132000/LConn1 -- _CN_199287768_500000_CN_193415212_132000/LConn1
  _CN_323007048_132000_CN_193415212_132000/RConn2 -- G_193415212_Central_Nuclear_de_Atucha_I/RConn2 -- 2ATVL1Y2_CN_277132135_220000_CN_193415212_132000/LConn2 -- _CN_193412175_500000_CN_193415212_132000/LConn2 -- _CN_199287768_500000_CN_193415212_132000/LConn2
  _CN_323007048_132000_CN_193415212_132000/RConn3 -- G_193415212_Central_Nuclear_de_Atucha_I/RConn3 -- 2ATVL1Y2_CN_277132135_220000_CN_193415212_132000/LConn3 -- _CN_193412175_500000_CN_193415212_132000/LConn3 -- _CN_199287768_500000_CN_193415212_132000/LConn3 -- bus122/LConn1
  T_321398721__/LConn1 -- _CN_321398723_132000_CN_321398721_132000/RConn1
  T_321398721__/LConn2 -- _CN_321398723_132000_CN_321398721_132000/RConn2
  _CN_321398723_132000_CN_321398721_132000/RConn3 -- T_321398721__/LConn3 -- bus123/LConn1
  T_259688907__/LConn1 -- _CN_259688907_132000_CN_230070479_132000/LConn1
  T_259688907__/LConn2 -- _CN_259688907_132000_CN_230070479_132000/LConn2
  _CN_259688907_132000_CN_230070479_132000/LConn3 -- T_259688907__/LConn3 -- bus124/LConn1
  G_230070479_Planta_Generadora_C_L_Y_F_E_M_A_/RConn1 -- _CN_259688907_132000_CN_230070479_132000/RConn1
  G_230070479_Planta_Generadora_C_L_Y_F_E_M_A_/RConn2 -- _CN_259688907_132000_CN_230070479_132000/RConn2
  _CN_259688907_132000_CN_230070479_132000/RConn3 -- G_230070479_Planta_Generadora_C_L_Y_F_E_M_A_/RConn3 -- bus125/LConn1
  _CN_203363075_220000_CN_179545958_220000/LConn1 -- T_203363075__/LConn1 -- _CN_203363075_220000_CN_431598950_220000/LConn1
  _CN_203363075_220000_CN_179545958_220000/LConn2 -- T_203363075__/LConn2 -- _CN_203363075_220000_CN_431598950_220000/LConn2
  _CN_203363075_220000_CN_179545958_220000/LConn3 -- T_203363075__/LConn3 -- _CN_203363075_220000_CN_431598950_220000/LConn3 -- bus126/LConn1
  _CN_203363075_220000_CN_179545958_220000/RConn1 -- T_179545958_500000_Estación_Transformadora_Ezeiza/RConn1 -- _CN_172440613_220000_CN_179545958_220000/LConn1 -- _CN_321398723_220000_CN_179545958_220000/LConn1 -- _CN_58676298_220000_CN_179545958_220000/LConn1
  _CN_203363075_220000_CN_179545958_220000/RConn2 -- T_179545958_500000_Estación_Transformadora_Ezeiza/RConn2 -- _CN_172440613_220000_CN_179545958_220000/LConn2 -- _CN_321398723_220000_CN_179545958_220000/LConn2 -- _CN_58676298_220000_CN_179545958_220000/LConn2
  _CN_203363075_220000_CN_179545958_220000/RConn3 -- T_179545958_500000_Estación_Transformadora_Ezeiza/RConn3 -- _CN_172440613_220000_CN_179545958_220000/LConn3 -- _CN_321398723_220000_CN_179545958_220000/LConn3 -- _CN_58676298_220000_CN_179545958_220000/LConn3 -- bus127/LConn1
  _CN_203363075_220000_CN_431598950_220000/RConn1 -- T_431598950__/LConn1 -- _CN_242365381_220000_CN_431598950_220000/LConn1
  _CN_203363075_220000_CN_431598950_220000/RConn2 -- T_431598950__/LConn2 -- _CN_242365381_220000_CN_431598950_220000/LConn2
  _CN_203363075_220000_CN_431598950_220000/RConn3 -- T_431598950__/LConn3 -- _CN_242365381_220000_CN_431598950_220000/LConn3 -- bus128/LConn1
  T_164577670__Estación_Electrica/LConn1 -- _CN_164577670_220000_CN_164673290_220000/LConn1
  T_164577670__Estación_Electrica/LConn2 -- _CN_164577670_220000_CN_164673290_220000/LConn2
  _CN_164577670_220000_CN_164673290_220000/LConn3 -- T_164577670__Estación_Electrica/LConn3 -- bus129/LConn1
  T_164673290__/LConn1 -- _CN_164577670_220000_CN_164673290_220000/RConn1
  T_164673290__/LConn2 -- _CN_164577670_220000_CN_164673290_220000/RConn2
  _CN_164577670_220000_CN_164673290_220000/RConn3 -- T_164673290__/LConn3 -- bus130/LConn1
  T_272051854__/LConn1 -- _CN_272051854_220000_CN_199287768_220000/LConn1
  T_272051854__/LConn2 -- _CN_272051854_220000_CN_199287768_220000/LConn2
  _CN_272051854_220000_CN_199287768_220000/LConn3 -- T_272051854__/LConn3 -- bus131/LConn1
  _CN_272051854_220000_CN_199287768_220000/RConn1 -- T_199287768_500000_Estación_Transformadora_General_Rodríguez/RConn1 -- _CN_199287768_220000_CN_277132135_220000/LConn1 -- L_199287768/LConn1 -- _CN_191859780_220000_CN_199287768_220000/LConn1
  _CN_272051854_220000_CN_199287768_220000/RConn2 -- T_199287768_500000_Estación_Transformadora_General_Rodríguez/RConn2 -- _CN_199287768_220000_CN_277132135_220000/LConn2 -- L_199287768/LConn2 -- _CN_191859780_220000_CN_199287768_220000/LConn2
  _CN_272051854_220000_CN_199287768_220000/RConn3 -- T_199287768_500000_Estación_Transformadora_General_Rodríguez/RConn3 -- _CN_199287768_220000_CN_277132135_220000/LConn3 -- L_199287768/LConn3 -- bus132/LConn1 -- _CN_191859780_220000_CN_199287768_220000/LConn3
  T_251673647__Subestación_La_Plata/LConn1 -- _CN_251673647_220000_CN_251081502_220000/LConn1
  T_251673647__Subestación_La_Plata/LConn2 -- _CN_251673647_220000_CN_251081502_220000/LConn2
  _CN_251673647_220000_CN_251081502_220000/LConn3 -- T_251673647__Subestación_La_Plata/LConn3 -- bus133/LConn1
  _CN_251673647_220000_CN_251081502_220000/RConn1 -- T_251081502_220000;500000_Estación_Transformadora_Abasto/RConn1 -- L_251081502/LConn1
  _CN_251673647_220000_CN_251081502_220000/RConn2 -- T_251081502_220000;500000_Estación_Transformadora_Abasto/RConn2 -- L_251081502/LConn2
  _CN_251673647_220000_CN_251081502_220000/RConn3 -- T_251081502_220000;500000_Estación_Transformadora_Abasto/RConn3 -- L_251081502/LConn3 -- bus134/LConn1
  T_273522974__/LConn1 -- _CN_273522974_220000_CN_285554517_220000/LConn1
  T_273522974__/LConn2 -- _CN_273522974_220000_CN_285554517_220000/LConn2
  _CN_273522974_220000_CN_285554517_220000/LConn3 -- T_273522974__/LConn3 -- bus135/LConn1
  _CN_273522974_220000_CN_285554517_220000/RConn1 -- T_285554517__/LConn1 -- _CN_285554517_220000_CN_285554522_220000/LConn1
  _CN_273522974_220000_CN_285554517_220000/RConn2 -- T_285554517__/LConn2 -- _CN_285554517_220000_CN_285554522_220000/LConn2
  _CN_273522974_220000_CN_285554517_220000/RConn3 -- T_285554517__/LConn3 -- _CN_285554517_220000_CN_285554522_220000/LConn3 -- bus136/LConn1
  T_172440613__/LConn1 -- _CN_172440613_220000_CN_179545958_220000/RConn1
  T_172440613__/LConn2 -- _CN_172440613_220000_CN_179545958_220000/RConn2
  _CN_172440613_220000_CN_179545958_220000/RConn3 -- T_172440613__/LConn3 -- bus137/LConn1
  _CN_193242927_220000_CN_191859780_220000/LConn1 -- T_193242927__/LConn1 -- _CN_193242927_220000_CN_178248568_220000/LConn1
  _CN_193242927_220000_CN_191859780_220000/LConn2 -- T_193242927__/LConn2 -- _CN_193242927_220000_CN_178248568_220000/LConn2
  _CN_193242927_220000_CN_191859780_220000/LConn3 -- T_193242927__/LConn3 -- _CN_193242927_220000_CN_178248568_220000/LConn3 -- bus138/LConn1
  _CN_193242927_220000_CN_191859780_220000/RConn1 -- T_191859780__/LConn1 -- _CN_191859780_220000_CN_199287768_220000/RConn1
  _CN_193242927_220000_CN_191859780_220000/RConn2 -- T_191859780__/LConn2 -- _CN_191859780_220000_CN_199287768_220000/RConn2
  _CN_193242927_220000_CN_191859780_220000/RConn3 -- T_191859780__/LConn3 -- _CN_191859780_220000_CN_199287768_220000/RConn3 -- bus139/LConn1
  _CN_193242927_220000_CN_178248568_220000/RConn1 -- T_178248568__/LConn1 -- _CN_310114524_220000_CN_178248568_220000/LConn1
  _CN_193242927_220000_CN_178248568_220000/RConn2 -- T_178248568__/LConn2 -- _CN_310114524_220000_CN_178248568_220000/LConn2
  _CN_193242927_220000_CN_178248568_220000/RConn3 -- T_178248568__/LConn3 -- _CN_310114524_220000_CN_178248568_220000/LConn3 -- bus140/LConn1
  T_321398723__/LConn1 -- _CN_321398723_220000_CN_179545958_220000/RConn1
  T_321398723__/LConn2 -- _CN_321398723_220000_CN_179545958_220000/RConn2
  _CN_321398723_220000_CN_179545958_220000/RConn3 -- T_321398723__/LConn3 -- bus141/LConn1
  T_242365381__/LConn1 -- _CN_242365381_220000_CN_431598950_220000/RConn1
  T_242365381__/LConn2 -- _CN_242365381_220000_CN_431598950_220000/RConn2
  _CN_242365381_220000_CN_431598950_220000/RConn3 -- T_242365381__/LConn3 -- bus142/LConn1
  T_58676298__Subestación_Edenor/LConn1 -- _CN_58676298_220000_CN_179545958_220000/RConn1
  T_58676298__Subestación_Edenor/LConn2 -- _CN_58676298_220000_CN_179545958_220000/RConn2
  _CN_58676298_220000_CN_179545958_220000/RConn3 -- T_58676298__Subestación_Edenor/LConn3 -- bus143/LConn1
  2RAVL1Y2_CN_193412175_220000_CN_277132135_220000/LConn1 -- T_193412175_500000_Estación_transformadora_Ramallo/RConn1 -- _CN_193412175_220000_CN_194378395_220000/LConn1
  2RAVL1Y2_CN_193412175_220000_CN_277132135_220000/LConn2 -- T_193412175_500000_Estación_transformadora_Ramallo/RConn2 -- _CN_193412175_220000_CN_194378395_220000/LConn2
  2RAVL1Y2_CN_193412175_220000_CN_277132135_220000/LConn3 -- T_193412175_500000_Estación_transformadora_Ramallo/RConn3 -- _CN_193412175_220000_CN_194378395_220000/LConn3 -- bus144/LConn1
  2RAVL1Y2_CN_193412175_220000_CN_277132135_220000/RConn1 -- T_277132135_220000_Estación_transformadora_Villa_Lía/LConn1 -- _CN_199287768_220000_CN_277132135_220000/RConn1 -- 2ATVL1Y2_CN_277132135_220000_CN_193415212_132000/RConn1
  2RAVL1Y2_CN_193412175_220000_CN_277132135_220000/RConn2 -- T_277132135_220000_Estación_transformadora_Villa_Lía/LConn2 -- _CN_199287768_220000_CN_277132135_220000/RConn2 -- 2ATVL1Y2_CN_277132135_220000_CN_193415212_132000/RConn2
  2RAVL1Y2_CN_193412175_220000_CN_277132135_220000/RConn3 -- T_277132135_220000_Estación_transformadora_Villa_Lía/LConn3 -- _CN_199287768_220000_CN_277132135_220000/RConn3 -- 2ATVL1Y2_CN_277132135_220000_CN_193415212_132000/RConn3 -- bus145/LConn1
  G_194378395_Argener/RConn1 -- _CN_193412175_220000_CN_194378395_220000/RConn1
  G_194378395_Argener/RConn2 -- _CN_193412175_220000_CN_194378395_220000/RConn2
  _CN_193412175_220000_CN_194378395_220000/RConn3 -- G_194378395_Argener/RConn3 -- bus146/LConn1
  G_285554522_Central_Eléctrica_Barragán/RConn1 -- _CN_285554517_220000_CN_285554522_220000/RConn1
  G_285554522_Central_Eléctrica_Barragán/RConn2 -- _CN_285554517_220000_CN_285554522_220000/RConn2
  _CN_285554517_220000_CN_285554522_220000/RConn3 -- G_285554522_Central_Eléctrica_Barragán/RConn3 -- bus147/LConn1
  T_310114524__Subestación_Edenor/LConn1 -- _CN_310114524_220000_CN_178248568_220000/RConn1
  T_310114524__Subestación_Edenor/LConn2 -- _CN_310114524_220000_CN_178248568_220000/RConn2
  _CN_310114524_220000_CN_178248568_220000/RConn3 -- T_310114524__Subestación_Edenor/LConn3 -- bus148/LConn1
  _CN_188360578_500000_CN_247830316_500000/LConn1 -- T_188360578__/LConn1 -- _CN_188360578_500000_CN_413038969_500000/LConn1
  _CN_188360578_500000_CN_247830316_500000/LConn2 -- T_188360578__/LConn2 -- _CN_188360578_500000_CN_413038969_500000/LConn2
  _CN_188360578_500000_CN_247830316_500000/LConn3 -- T_188360578__/LConn3 -- _CN_188360578_500000_CN_413038969_500000/LConn3 -- bus149/LConn1
  _CN_188360578_500000_CN_247830316_500000/RConn1 -- T_247830316__/LConn1 -- _CN_247830316_500000_CN_218457595_500000/LConn1 -- _CN_247830316_500000_CN_176046623_500000/LConn1
  _CN_188360578_500000_CN_247830316_500000/RConn2 -- T_247830316__/LConn2 -- _CN_247830316_500000_CN_218457595_500000/LConn2 -- _CN_247830316_500000_CN_176046623_500000/LConn2
  _CN_188360578_500000_CN_247830316_500000/RConn3 -- T_247830316__/LConn3 -- _CN_247830316_500000_CN_218457595_500000/LConn3 -- bus150/LConn1 -- _CN_247830316_500000_CN_176046623_500000/LConn3
  _CN_188360578_500000_CN_413038969_500000/RConn1 -- T_413038969__/LConn1 -- _CN_26119134_500000_CN_413038969_500000/LConn1 -- _CN_413038969_500000_CN_178480305_500000/LConn1 -- _CN_213192904_500000_CN_413038969_500000/LConn1
  _CN_188360578_500000_CN_413038969_500000/RConn2 -- T_413038969__/LConn2 -- _CN_26119134_500000_CN_413038969_500000/LConn2 -- _CN_413038969_500000_CN_178480305_500000/LConn2 -- _CN_213192904_500000_CN_413038969_500000/LConn2
  _CN_188360578_500000_CN_413038969_500000/RConn3 -- T_413038969__/LConn3 -- _CN_26119134_500000_CN_413038969_500000/LConn3 -- _CN_413038969_500000_CN_178480305_500000/LConn3 -- bus151/LConn1 -- _CN_213192904_500000_CN_413038969_500000/LConn3
  _CN_277426564_500000_CN_277641813_500000/LConn1 -- T_277426564__/LConn1 -- _CN_277426564_500000_CN_251081502_500000/LConn1
  _CN_277426564_500000_CN_277641813_500000/LConn2 -- T_277426564__/LConn2 -- _CN_277426564_500000_CN_251081502_500000/LConn2
  _CN_277426564_500000_CN_277641813_500000/LConn3 -- T_277426564__/LConn3 -- _CN_277426564_500000_CN_251081502_500000/LConn3 -- bus152/LConn1
  _CN_277426564_500000_CN_277641813_500000/RConn1 -- T_277641813__/LConn1 -- _CN_71775909_500000_CN_277641813_500000/LConn1 -- _CN_277641813_500000_CN_26119134_500000/LConn1
  _CN_277426564_500000_CN_277641813_500000/RConn2 -- T_277641813__/LConn2 -- _CN_71775909_500000_CN_277641813_500000/LConn2 -- _CN_277641813_500000_CN_26119134_500000/LConn2
  _CN_277426564_500000_CN_277641813_500000/RConn3 -- T_277641813__/LConn3 -- _CN_71775909_500000_CN_277641813_500000/LConn3 -- _CN_277641813_500000_CN_26119134_500000/LConn3 -- bus153/LConn1
  _CN_277426564_500000_CN_251081502_500000/RConn1 -- T_251081502_220000;500000_Estación_Transformadora_Abasto/LConn1 -- _CN_251081502_500000_CN_179545958_500000/LConn1
  _CN_277426564_500000_CN_251081502_500000/RConn2 -- T_251081502_220000;500000_Estación_Transformadora_Abasto/LConn2 -- _CN_251081502_500000_CN_179545958_500000/LConn2
  _CN_277426564_500000_CN_251081502_500000/RConn3 -- T_251081502_220000;500000_Estación_Transformadora_Abasto/LConn3 -- _CN_251081502_500000_CN_179545958_500000/LConn3 -- bus154/LConn1
  _CN_247830316_500000_CN_176046623_500000/RConn1 -- T_176046623__/LConn1 -- _CN_176046623_500000_CN_247830317_500000/LConn1
  _CN_247830316_500000_CN_176046623_500000/RConn2 -- T_176046623__/LConn2 -- _CN_176046623_500000_CN_247830317_500000/LConn2
  _CN_247830316_500000_CN_176046623_500000/RConn3 -- T_176046623__/LConn3 -- _CN_176046623_500000_CN_247830317_500000/LConn3 -- bus155/LConn1
  T_218457595__/LConn1 -- _CN_247830316_500000_CN_218457595_500000/RConn1
  T_218457595__/LConn2 -- _CN_247830316_500000_CN_218457595_500000/RConn2
  _CN_247830316_500000_CN_218457595_500000/RConn3 -- T_218457595__/LConn3 -- bus156/LConn1
  _CN_110339851_500000_CN_258696364_500000/LConn1 -- T_110339851__Estación_Transformadora_Puerto_Bastiani/LConn1 -- _CN_110339851_500000_CN_305162903_500000/LConn1 -- _CN_110339851_500000_CN_258696366_500000/LConn1
  _CN_110339851_500000_CN_258696364_500000/LConn2 -- T_110339851__Estación_Transformadora_Puerto_Bastiani/LConn2 -- _CN_110339851_500000_CN_305162903_500000/LConn2 -- _CN_110339851_500000_CN_258696366_500000/LConn2
  _CN_110339851_500000_CN_258696364_500000/LConn3 -- T_110339851__Estación_Transformadora_Puerto_Bastiani/LConn3 -- _CN_110339851_500000_CN_305162903_500000/LConn3 -- bus157/LConn1 -- _CN_110339851_500000_CN_258696366_500000/LConn3
  _CN_110339851_500000_CN_258696364_500000/RConn1 -- T_258696364__/LConn1 -- _CN_258696364_500000_CN_221357412_500000/LConn1
  _CN_110339851_500000_CN_258696364_500000/RConn2 -- T_258696364__/LConn2 -- _CN_258696364_500000_CN_221357412_500000/LConn2
  _CN_110339851_500000_CN_258696364_500000/RConn3 -- T_258696364__/LConn3 -- _CN_258696364_500000_CN_221357412_500000/LConn3 -- bus158/LConn1
  _CN_110339851_500000_CN_258696366_500000/RConn1 -- T_258696366__/LConn1 -- _CN_305027751_500000_CN_258696366_500000/LConn1
  _CN_110339851_500000_CN_258696366_500000/RConn2 -- T_258696366__/LConn2 -- _CN_305027751_500000_CN_258696366_500000/LConn2
  _CN_110339851_500000_CN_258696366_500000/RConn3 -- T_258696366__/LConn3 -- _CN_305027751_500000_CN_258696366_500000/LConn3 -- bus159/LConn1
  T_305162903__/LConn1 -- _CN_110339851_500000_CN_305162903_500000/RConn1
  T_305162903__/LConn2 -- _CN_110339851_500000_CN_305162903_500000/RConn2
  _CN_110339851_500000_CN_305162903_500000/RConn3 -- T_305162903__/LConn3 -- bus160/LConn1
  _CN_203954946_500000_CN_190845501_500000/LConn1 -- T_203954946_500000_Estación_transformadora_Colonia_Elía/LConn1 -- _CN_203954946_500000_CN_274067533_500000/LConn1 -- _CN_203954946_500000_CN_186421221_500000/LConn1 -- _CN_203954946_500000_CN_199287768_500000/LConn1
  _CN_203954946_500000_CN_190845501_500000/LConn2 -- T_203954946_500000_Estación_transformadora_Colonia_Elía/LConn2 -- _CN_203954946_500000_CN_274067533_500000/LConn2 -- _CN_203954946_500000_CN_186421221_500000/LConn2 -- _CN_203954946_500000_CN_199287768_500000/LConn2
  _CN_203954946_500000_CN_190845501_500000/LConn3 -- T_203954946_500000_Estación_transformadora_Colonia_Elía/LConn3 -- _CN_203954946_500000_CN_274067533_500000/LConn3 -- _CN_203954946_500000_CN_186421221_500000/LConn3 -- _CN_203954946_500000_CN_199287768_500000/LConn3 -- bus161/LConn1
  T_190845501__/LConn1 -- _CN_203954946_500000_CN_190845501_500000/RConn1
  T_190845501__/LConn2 -- _CN_203954946_500000_CN_190845501_500000/RConn2
  _CN_203954946_500000_CN_190845501_500000/RConn3 -- T_190845501__/LConn3 -- bus162/LConn1
  _CN_203954946_500000_CN_274067533_500000/RConn1 -- T_274067533__/LConn1 -- _CN_274067533_500000_CN_221357412_500000/LConn1
  _CN_203954946_500000_CN_274067533_500000/RConn2 -- T_274067533__/LConn2 -- _CN_274067533_500000_CN_221357412_500000/LConn2
  _CN_203954946_500000_CN_274067533_500000/RConn3 -- T_274067533__/LConn3 -- _CN_274067533_500000_CN_221357412_500000/LConn3 -- bus163/LConn1
  _CN_203954946_500000_CN_186421221_500000/RConn1 -- T_186421221__/LConn1 -- _CN_305027751_500000_CN_186421221_500000/LConn1 -- _CN_221357412_500000_CN_186421221_500000/LConn1
  _CN_203954946_500000_CN_186421221_500000/RConn2 -- T_186421221__/LConn2 -- _CN_305027751_500000_CN_186421221_500000/LConn2 -- _CN_221357412_500000_CN_186421221_500000/LConn2
  _CN_203954946_500000_CN_186421221_500000/RConn3 -- T_186421221__/LConn3 -- _CN_305027751_500000_CN_186421221_500000/LConn3 -- _CN_221357412_500000_CN_186421221_500000/LConn3 -- bus164/LConn1
  _CN_203954946_500000_CN_199287768_500000/RConn1 -- T_199287768_500000_Estación_Transformadora_General_Rodríguez/LConn1 -- _CN_215284908_500000_CN_199287768_500000/LConn1 -- _CN_199287768_500000_CN_193415212_132000/RConn1 -- _CN_199287768_500000_CN_179545958_500000/LConn1
  _CN_203954946_500000_CN_199287768_500000/RConn2 -- T_199287768_500000_Estación_Transformadora_General_Rodríguez/LConn2 -- _CN_215284908_500000_CN_199287768_500000/LConn2 -- _CN_199287768_500000_CN_193415212_132000/RConn2 -- _CN_199287768_500000_CN_179545958_500000/LConn2
  _CN_203954946_500000_CN_199287768_500000/RConn3 -- T_199287768_500000_Estación_Transformadora_General_Rodríguez/LConn3 -- _CN_215284908_500000_CN_199287768_500000/LConn3 -- _CN_199287768_500000_CN_193415212_132000/RConn3 -- _CN_199287768_500000_CN_179545958_500000/LConn3 -- bus165/LConn1
  T_247820688__/LConn1 -- _CN_247820688_500000_CN_89373622_500000/LConn1
  T_247820688__/LConn2 -- _CN_247820688_500000_CN_89373622_500000/LConn2
  _CN_247820688_500000_CN_89373622_500000/LConn3 -- T_247820688__/LConn3 -- bus166/LConn1
  T_89373622__/LConn1 -- _CN_247820688_500000_CN_89373622_500000/RConn1
  T_89373622__/LConn2 -- _CN_247820688_500000_CN_89373622_500000/RConn2
  _CN_247820688_500000_CN_89373622_500000/RConn3 -- T_89373622__/LConn3 -- bus167/LConn1
  _CN_257673618_500000_CN_179545958_500000/LConn1 -- T_257673618__/LConn1 -- _CN_257673618_500000_CN_247830317_500000/LConn1
  _CN_257673618_500000_CN_179545958_500000/LConn2 -- T_257673618__/LConn2 -- _CN_257673618_500000_CN_247830317_500000/LConn2
  _CN_257673618_500000_CN_179545958_500000/LConn3 -- T_257673618__/LConn3 -- _CN_257673618_500000_CN_247830317_500000/LConn3 -- bus168/LConn1
  _CN_257673618_500000_CN_179545958_500000/RConn1 -- T_179545958_500000_Estación_Transformadora_Ezeiza/LConn1 -- _CN_251081502_500000_CN_179545958_500000/RConn1 -- _CN_199287768_500000_CN_179545958_500000/RConn1
  _CN_257673618_500000_CN_179545958_500000/RConn2 -- T_179545958_500000_Estación_Transformadora_Ezeiza/LConn2 -- _CN_251081502_500000_CN_179545958_500000/RConn2 -- _CN_199287768_500000_CN_179545958_500000/RConn2
  _CN_257673618_500000_CN_179545958_500000/RConn3 -- T_179545958_500000_Estación_Transformadora_Ezeiza/LConn3 -- _CN_251081502_500000_CN_179545958_500000/RConn3 -- _CN_199287768_500000_CN_179545958_500000/RConn3 -- bus169/LConn1
  _CN_257673618_500000_CN_247830317_500000/RConn1 -- T_247830317__/LConn1 -- _CN_176046623_500000_CN_247830317_500000/RConn1
  _CN_257673618_500000_CN_247830317_500000/RConn2 -- T_247830317__/LConn2 -- _CN_176046623_500000_CN_247830317_500000/RConn2
  _CN_257673618_500000_CN_247830317_500000/RConn3 -- T_247830317__/LConn3 -- _CN_176046623_500000_CN_247830317_500000/RConn3 -- bus170/LConn1
  _CN_194575899_500000_CN_213568638_500000/LConn1 -- T_194575899__/LConn1 -- _CN_194575899_500000_CN_213353516_132000/RConn1
  _CN_194575899_500000_CN_213568638_500000/LConn2 -- T_194575899__/LConn2 -- _CN_194575899_500000_CN_213353516_132000/RConn2
  _CN_194575899_500000_CN_213568638_500000/LConn3 -- T_194575899__/LConn3 -- _CN_194575899_500000_CN_213353516_132000/RConn3 -- bus171/LConn1
  _CN_194575899_500000_CN_213568638_500000/RConn1 -- T_213568638__/LConn1 -- _CN_305103437_500000_CN_213568638_500000/LConn1
  _CN_194575899_500000_CN_213568638_500000/RConn2 -- T_213568638__/LConn2 -- _CN_305103437_500000_CN_213568638_500000/LConn2
  _CN_194575899_500000_CN_213568638_500000/RConn3 -- T_213568638__/LConn3 -- _CN_305103437_500000_CN_213568638_500000/LConn3 -- bus172/LConn1
  T_71775909__Central_Termoeléctrica_Piedra_Buena/LConn1 -- _CN_71775909_500000_CN_277641813_500000/RConn1
  T_71775909__Central_Termoeléctrica_Piedra_Buena/LConn2 -- _CN_71775909_500000_CN_277641813_500000/RConn2
  _CN_71775909_500000_CN_277641813_500000/RConn3 -- T_71775909__Central_Termoeléctrica_Piedra_Buena/LConn3 -- bus173/LConn1
  _CN_305027751_500000_CN_258696366_500000/RConn1 -- T_305027751__/LConn1 -- _CN_305027751_500000_CN_186421221_500000/RConn1
  _CN_305027751_500000_CN_258696366_500000/RConn2 -- T_305027751__/LConn2 -- _CN_305027751_500000_CN_186421221_500000/RConn2
  _CN_305027751_500000_CN_258696366_500000/RConn3 -- T_305027751__/LConn3 -- _CN_305027751_500000_CN_186421221_500000/RConn3 -- bus174/LConn1
  T_215284908_500000_Estación_Transformadora_Manuel_Belgrano/LConn1 -- _CN_215284908_500000_CN_199287768_500000/RConn1
  T_215284908_500000_Estación_Transformadora_Manuel_Belgrano/LConn2 -- _CN_215284908_500000_CN_199287768_500000/RConn2
  _CN_215284908_500000_CN_199287768_500000/RConn3 -- T_215284908_500000_Estación_Transformadora_Manuel_Belgrano/LConn3 -- bus175/LConn1
  _CN_213578175_500000_CN_213353516_132000/RConn1 -- T_213578175__Subestación_eléctrica/LConn1 -- _CN_213578175_500000_CN_253226994_500000/LConn1
  _CN_213578175_500000_CN_213353516_132000/RConn2 -- T_213578175__Subestación_eléctrica/LConn2 -- _CN_213578175_500000_CN_253226994_500000/LConn2
  _CN_213578175_500000_CN_213353516_132000/RConn3 -- T_213578175__Subestación_eléctrica/LConn3 -- _CN_213578175_500000_CN_253226994_500000/LConn3 -- bus176/LConn1
  _CN_213578175_500000_CN_253226994_500000/RConn1 -- T_253226994__/LConn1 -- _CN_173947403_500000_CN_253226994_500000/LConn1
  _CN_213578175_500000_CN_253226994_500000/RConn2 -- T_253226994__/LConn2 -- _CN_173947403_500000_CN_253226994_500000/LConn2
  _CN_213578175_500000_CN_253226994_500000/RConn3 -- T_253226994__/LConn3 -- _CN_173947403_500000_CN_253226994_500000/LConn3 -- bus177/LConn1
  _CN_314753857_500000_CN_314176103_500000/LConn1 -- T_314753857__Estación_transformadora_Piedrabuena/LConn1 -- _CN_314753857_500000_CN_303134158_500000/LConn1
  _CN_314753857_500000_CN_314176103_500000/LConn2 -- T_314753857__Estación_transformadora_Piedrabuena/LConn2 -- _CN_314753857_500000_CN_303134158_500000/LConn2
  _CN_314753857_500000_CN_314176103_500000/LConn3 -- T_314753857__Estación_transformadora_Piedrabuena/LConn3 -- _CN_314753857_500000_CN_303134158_500000/LConn3 -- bus178/LConn1
  T_314176103__Estación_transformadora_Esperanza/LConn1 -- _CN_314753857_500000_CN_314176103_500000/RConn1
  T_314176103__Estación_transformadora_Esperanza/LConn2 -- _CN_314753857_500000_CN_314176103_500000/RConn2
  _CN_314753857_500000_CN_314176103_500000/RConn3 -- T_314176103__Estación_transformadora_Esperanza/LConn3 -- bus179/LConn1
  _CN_314753857_500000_CN_303134158_500000/RConn1 -- T_303134158__/LConn1 -- _CN_303134158_500000_CN_26119134_500000/LConn1
  _CN_314753857_500000_CN_303134158_500000/RConn2 -- T_303134158__/LConn2 -- _CN_303134158_500000_CN_26119134_500000/LConn2
  _CN_314753857_500000_CN_303134158_500000/RConn3 -- T_303134158__/LConn3 -- _CN_303134158_500000_CN_26119134_500000/LConn3 -- bus180/LConn1
  _CN_173947403_500000_CN_253226994_500000/RConn1 -- T_173947403__Transener_S_A_/LConn1 -- 5GMRDI1_CN_173947403_500000_CN_306717418_500000/LConn1
  _CN_173947403_500000_CN_253226994_500000/RConn2 -- T_173947403__Transener_S_A_/LConn2 -- 5GMRDI1_CN_173947403_500000_CN_306717418_500000/LConn2
  _CN_173947403_500000_CN_253226994_500000/RConn3 -- T_173947403__Transener_S_A_/LConn3 -- 5GMRDI1_CN_173947403_500000_CN_306717418_500000/LConn3 -- bus181/LConn1
  5GMRDI1_CN_173947403_500000_CN_306717418_500000/RConn1 -- T_306717418__/LConn1 -- 5ECORDI1_CN_306717418_500000_CN_178480305_500000/LConn1
  5GMRDI1_CN_173947403_500000_CN_306717418_500000/RConn2 -- T_306717418__/LConn2 -- 5ECORDI1_CN_306717418_500000_CN_178480305_500000/LConn2
  5GMRDI1_CN_173947403_500000_CN_306717418_500000/RConn3 -- T_306717418__/LConn3 -- 5ECORDI1_CN_306717418_500000_CN_178480305_500000/LConn3 -- bus182/LConn1
  _CN_213192902_500000_CN_213192904_500000/LConn1 -- T_213192902__/LConn1 -- _CN_213192902_500000_CN_213192903_500000/LConn1
  _CN_213192902_500000_CN_213192904_500000/LConn2 -- T_213192902__/LConn2 -- _CN_213192902_500000_CN_213192903_500000/LConn2
  _CN_213192902_500000_CN_213192904_500000/LConn3 -- T_213192902__/LConn3 -- _CN_213192902_500000_CN_213192903_500000/LConn3 -- bus183/LConn1
  _CN_213192902_500000_CN_213192904_500000/RConn1 -- T_213192904__/LConn1 -- _CN_213192904_500000_CN_26119134_500000/LConn1 -- _CN_213192904_500000_CN_279914161_500000/LConn1 -- _CN_213192904_500000_CN_413038969_500000/RConn1
  _CN_213192902_500000_CN_213192904_500000/RConn2 -- T_213192904__/LConn2 -- _CN_213192904_500000_CN_26119134_500000/LConn2 -- _CN_213192904_500000_CN_279914161_500000/LConn2 -- _CN_213192904_500000_CN_413038969_500000/RConn2
  _CN_213192902_500000_CN_213192904_500000/RConn3 -- T_213192904__/LConn3 -- _CN_213192904_500000_CN_26119134_500000/LConn3 -- _CN_213192904_500000_CN_279914161_500000/LConn3 -- bus184/LConn1 -- _CN_213192904_500000_CN_413038969_500000/RConn3
  T_213192903__/LConn1 -- _CN_213192902_500000_CN_213192903_500000/RConn1
  T_213192903__/LConn2 -- _CN_213192902_500000_CN_213192903_500000/RConn2
  _CN_213192902_500000_CN_213192903_500000/RConn3 -- T_213192903__/LConn3 -- bus185/LConn1
  _CN_213192904_500000_CN_26119134_500000/RConn1 -- T_26119134__Transener_S_A_/LConn1 -- _CN_26119134_500000_CN_413038969_500000/RConn1 -- _CN_277641813_500000_CN_26119134_500000/RConn1 -- _CN_303134158_500000_CN_26119134_500000/RConn1
  _CN_213192904_500000_CN_26119134_500000/RConn2 -- T_26119134__Transener_S_A_/LConn2 -- _CN_26119134_500000_CN_413038969_500000/RConn2 -- _CN_277641813_500000_CN_26119134_500000/RConn2 -- _CN_303134158_500000_CN_26119134_500000/RConn2
  _CN_213192904_500000_CN_26119134_500000/RConn3 -- T_26119134__Transener_S_A_/LConn3 -- _CN_26119134_500000_CN_413038969_500000/RConn3 -- bus186/LConn1 -- _CN_277641813_500000_CN_26119134_500000/RConn3 -- _CN_303134158_500000_CN_26119134_500000/RConn3
  G_279914161_Hidroeléctrica_Pichi_Picún_Leufú/RConn1 -- _CN_213192904_500000_CN_279914161_500000/RConn1
  G_279914161_Hidroeléctrica_Pichi_Picún_Leufú/RConn2 -- _CN_213192904_500000_CN_279914161_500000/RConn2
  _CN_213192904_500000_CN_279914161_500000/RConn3 -- G_279914161_Hidroeléctrica_Pichi_Picún_Leufú/RConn3 -- bus187/LConn1
  _CN_274067533_500000_CN_221357412_500000/RConn1 -- T_221357412__Central_Hidroeléctrica_de_Yacyretá_Apipé/LConn1 -- _CN_221357412_500000_CN_204484095_500000/LConn1 -- _CN_258696364_500000_CN_221357412_500000/RConn1 -- _CN_221357412_500000_CN_186421221_500000/RConn1
  _CN_274067533_500000_CN_221357412_500000/RConn2 -- T_221357412__Central_Hidroeléctrica_de_Yacyretá_Apipé/LConn2 -- _CN_221357412_500000_CN_204484095_500000/LConn2 -- _CN_258696364_500000_CN_221357412_500000/RConn2 -- _CN_221357412_500000_CN_186421221_500000/RConn2
  _CN_274067533_500000_CN_221357412_500000/RConn3 -- T_221357412__Central_Hidroeléctrica_de_Yacyretá_Apipé/LConn3 -- _CN_221357412_500000_CN_204484095_500000/LConn3 -- bus188/LConn1 -- _CN_258696364_500000_CN_221357412_500000/RConn3 -- _CN_221357412_500000_CN_186421221_500000/RConn3
  _CN_193412175_500000_CN_323007074_500000/LConn1 -- T_193412175_500000_Estación_transformadora_Ramallo/LConn1 -- _CN_193412175_500000_CN_193415212_132000/RConn1
  _CN_193412175_500000_CN_323007074_500000/LConn2 -- T_193412175_500000_Estación_transformadora_Ramallo/LConn2 -- _CN_193412175_500000_CN_193415212_132000/RConn2
  _CN_193412175_500000_CN_323007074_500000/LConn3 -- T_193412175_500000_Estación_transformadora_Ramallo/LConn3 -- _CN_193412175_500000_CN_193415212_132000/RConn3 -- bus189/LConn1
  T_323007074__/LConn1 -- _CN_193412175_500000_CN_323007074_500000/RConn1
  T_323007074__/LConn2 -- _CN_193412175_500000_CN_323007074_500000/RConn2
  _CN_193412175_500000_CN_323007074_500000/RConn3 -- T_323007074__/LConn3 -- bus190/LConn1
  T_305103439__/LConn1 -- _CN_305103439_500000_CN_305103437_500000/LConn1
  T_305103439__/LConn2 -- _CN_305103439_500000_CN_305103437_500000/LConn2
  _CN_305103439_500000_CN_305103437_500000/LConn3 -- T_305103439__/LConn3 -- bus191/LConn1
  _CN_305103439_500000_CN_305103437_500000/RConn1 -- T_305103437__/LConn1 -- _CN_305103437_500000_CN_213568638_500000/RConn1
  _CN_305103439_500000_CN_305103437_500000/RConn2 -- T_305103437__/LConn2 -- _CN_305103437_500000_CN_213568638_500000/RConn2
  _CN_305103439_500000_CN_305103437_500000/RConn3 -- T_305103437__/LConn3 -- _CN_305103437_500000_CN_213568638_500000/RConn3 -- bus192/LConn1
  T_204484095__/LConn1 -- _CN_221357412_500000_CN_204484095_500000/RConn1
  T_204484095__/LConn2 -- _CN_221357412_500000_CN_204484095_500000/RConn2
  _CN_221357412_500000_CN_204484095_500000/RConn3 -- T_204484095__/LConn3 -- bus193/LConn1
  5ECORDI1_CN_306717418_500000_CN_178480305_500000/RConn1 -- G_178480305_Central_Termoeléctrica/RConn1 -- _CN_413038969_500000_CN_178480305_500000/RConn1
  5ECORDI1_CN_306717418_500000_CN_178480305_500000/RConn2 -- G_178480305_Central_Termoeléctrica/RConn2 -- _CN_413038969_500000_CN_178480305_500000/RConn2
  5ECORDI1_CN_306717418_500000_CN_178480305_500000/RConn3 -- G_178480305_Central_Termoeléctrica/RConn3 -- _CN_413038969_500000_CN_178480305_500000/RConn3 -- bus194/LConn1
  T_413160960__/RConn1 -- L_413160960/LConn1
  T_413160960__/RConn2 -- L_413160960/LConn2
  L_413160960/LConn3 -- T_413160960__/RConn3 -- bus195/LConn1
  T_413160965__/RConn1 -- L_413160965/LConn1
  T_413160965__/RConn2 -- L_413160965/LConn2
  L_413160965/LConn3 -- T_413160965__/RConn3 -- bus196/LConn1
  T_124680196__/RConn1 -- L_124680196/LConn1
  T_124680196__/RConn2 -- L_124680196/LConn2
  L_124680196/LConn3 -- T_124680196__/RConn3 -- bus197/LConn1
  T_429400926_132000_Estación_Parque_eólico_Loma_Blanca/RConn1 -- L_429400926/LConn1
  T_429400926_132000_Estación_Parque_eólico_Loma_Blanca/RConn2 -- L_429400926/LConn2
  L_429400926/LConn3 -- T_429400926_132000_Estación_Parque_eólico_Loma_Blanca/RConn3 -- bus198/LConn1
  T_313124869__/RConn1 -- L_313124869/LConn1
  T_313124869__/RConn2 -- L_313124869/LConn2
  L_313124869/LConn3 -- T_313124869__/RConn3 -- bus199/LConn1
  T_323007043__/RConn1 -- L_323007043/LConn1
  T_323007043__/RConn2 -- L_323007043/LConn2
  L_323007043/LConn3 -- T_323007043__/RConn3 -- bus200/LConn1
  T_193433094__Estación_transformadora_Santa_Cruz_Norte/RConn1 -- L_193433094/LConn1
  T_193433094__Estación_transformadora_Santa_Cruz_Norte/RConn2 -- L_193433094/LConn2
  L_193433094/LConn3 -- T_193433094__Estación_transformadora_Santa_Cruz_Norte/RConn3 -- bus201/LConn1
  T_299759041__Subestación_transformadora_San_José/RConn1 -- L_299759041/LConn1
  T_299759041__Subestación_transformadora_San_José/RConn2 -- L_299759041/LConn2
  L_299759041/LConn3 -- T_299759041__Subestación_transformadora_San_José/RConn3 -- bus202/LConn1
  T_413160968__/RConn1 -- L_413160968/LConn1
  T_413160968__/RConn2 -- L_413160968/LConn2
  L_413160968/LConn3 -- T_413160968__/RConn3 -- bus203/LConn1
  T_400351708__Estación_transformadora_Pergamino/RConn1 -- L_400351708/LConn1
  T_400351708__Estación_transformadora_Pergamino/RConn2 -- L_400351708/LConn2
  L_400351708/LConn3 -- T_400351708__Estación_transformadora_Pergamino/RConn3 -- bus204/LConn1
  T_413160970__/RConn1 -- L_413160970/LConn1
  T_413160970__/RConn2 -- L_413160970/LConn2
  L_413160970/LConn3 -- T_413160970__/RConn3 -- bus205/LConn1
  T_215284916_500000_Estación_Transformadora_Campana/RConn1 -- L_215284916/LConn1
  T_215284916_500000_Estación_Transformadora_Campana/RConn2 -- L_215284916/LConn2
  L_215284916/LConn3 -- T_215284916_500000_Estación_Transformadora_Campana/RConn3 -- bus206/LConn1
  T_321753613__/RConn1 -- L_321753613/LConn1
  T_321753613__/RConn2 -- L_321753613/LConn2
  L_321753613/LConn3 -- T_321753613__/RConn3 -- bus207/LConn1
  T_274188832__/RConn1 -- L_274188832/LConn1
  T_274188832__/RConn2 -- L_274188832/LConn2
  L_274188832/LConn3 -- T_274188832__/RConn3 -- bus208/LConn1
  T_208412024__Eléctrica/RConn1 -- L_208412024/LConn1
  T_208412024__Eléctrica/RConn2 -- L_208412024/LConn2
  L_208412024/LConn3 -- T_208412024__Eléctrica/RConn3 -- bus209/LConn1
  T_263644686__/RConn1 -- L_263644686/LConn1
  T_263644686__/RConn2 -- L_263644686/LConn2
  L_263644686/LConn3 -- T_263644686__/RConn3 -- bus210/LConn1
  T_254366935__/RConn1 -- L_254366935/LConn1
  T_254366935__/RConn2 -- L_254366935/LConn2
  L_254366935/LConn3 -- T_254366935__/RConn3 -- bus211/LConn1
  T_348404653__/RConn1 -- L_348404653/LConn1
  T_348404653__/RConn2 -- L_348404653/LConn2
  L_348404653/LConn3 -- T_348404653__/RConn3 -- bus212/LConn1
  T_348413858__/RConn1 -- L_348413858/LConn1
  T_348413858__/RConn2 -- L_348413858/LConn2
  L_348413858/LConn3 -- T_348413858__/RConn3 -- bus213/LConn1
  T_413160978__/RConn1 -- L_413160978/LConn1
  T_413160978__/RConn2 -- L_413160978/LConn2
  L_413160978/LConn3 -- T_413160978__/RConn3 -- bus214/LConn1
  T_413160933__/RConn1 -- L_413160933/LConn1
  T_413160933__/RConn2 -- L_413160933/LConn2
  L_413160933/LConn3 -- T_413160933__/RConn3 -- bus215/LConn1
  T_314578968_132000_/RConn1 -- L_314578968/LConn1
  T_314578968_132000_/RConn2 -- L_314578968/LConn2
  L_314578968/LConn3 -- T_314578968_132000_/RConn3 -- bus216/LConn1
  T_267158870__/RConn1 -- L_267158870/LConn1
  T_267158870__/RConn2 -- L_267158870/LConn2
  L_267158870/LConn3 -- T_267158870__/RConn3 -- bus217/LConn1
  T_277641812__/RConn1 -- L_277641812/LConn1
  T_277641812__/RConn2 -- L_277641812/LConn2
  L_277641812/LConn3 -- T_277641812__/RConn3 -- bus218/LConn1
  T_276036475__/RConn1 -- L_276036475/LConn1
  T_276036475__/RConn2 -- L_276036475/LConn2
  L_276036475/LConn3 -- T_276036475__/RConn3 -- bus219/LConn1
  T_277739296_132000_/RConn1 -- L_277739296/LConn1
  T_277739296_132000_/RConn2 -- L_277739296/LConn2
  L_277739296/LConn3 -- T_277739296_132000_/RConn3 -- bus220/LConn1
  T_329781274__/RConn1 -- L_329781274/LConn1
  T_329781274__/RConn2 -- L_329781274/LConn2
  L_329781274/LConn3 -- T_329781274__/RConn3 -- bus221/LConn1
  T_188145045__/RConn1 -- L_188145045/LConn1
  T_188145045__/RConn2 -- L_188145045/LConn2
  L_188145045/LConn3 -- T_188145045__/RConn3 -- bus222/LConn1
  T_193707888__/RConn1 -- L_193707888/LConn1
  T_193707888__/RConn2 -- L_193707888/LConn2
  L_193707888/LConn3 -- T_193707888__/RConn3 -- bus223/LConn1
  T_230950275__/RConn1 -- L_230950275/LConn1
  T_230950275__/RConn2 -- L_230950275/LConn2
  L_230950275/LConn3 -- T_230950275__/RConn3 -- bus224/LConn1
  T_214867294__/RConn1 -- L_214867294/LConn1
  T_214867294__/RConn2 -- L_214867294/LConn2
  L_214867294/LConn3 -- T_214867294__/RConn3 -- bus225/LConn1
  T_251640352__Subestación_Sudeste/RConn1 -- L_251640352/LConn1
  T_251640352__Subestación_Sudeste/RConn2 -- L_251640352/LConn2
  L_251640352/LConn3 -- T_251640352__Subestación_Sudeste/RConn3 -- bus226/LConn1
  T_320719910__/RConn1 -- L_320719910/LConn1
  T_320719910__/RConn2 -- L_320719910/LConn2
  L_320719910/LConn3 -- T_320719910__/RConn3 -- bus227/LConn1
  T_323007038__/RConn1 -- L_323007038/LConn1
  T_323007038__/RConn2 -- L_323007038/LConn2
  L_323007038/LConn3 -- T_323007038__/RConn3 -- bus228/LConn1
  T_381521453__/RConn1 -- L_381521453/LConn1
  T_381521453__/RConn2 -- L_381521453/LConn2
  L_381521453/LConn3 -- T_381521453__/RConn3 -- bus229/LConn1
  T_323007048__/RConn1 -- L_323007048/LConn1
  T_323007048__/RConn2 -- L_323007048/LConn2
  L_323007048/LConn3 -- T_323007048__/RConn3 -- bus230/LConn1
  T_199147054_132000_Estación_Transformadora_Malvinas/RConn1 -- L_199147054/LConn1
  T_199147054_132000_Estación_Transformadora_Malvinas/RConn2 -- L_199147054/LConn2
  L_199147054/LConn3 -- T_199147054_132000_Estación_Transformadora_Malvinas/RConn3 -- bus231/LConn1
  T_195246048__/RConn1 -- L_195246048/LConn1
  T_195246048__/RConn2 -- L_195246048/LConn2
  L_195246048/LConn3 -- T_195246048__/RConn3 -- bus232/LConn1
  T_285751980_132000_Estación_Transformadora_Luján/RConn1 -- L_285751980/LConn1
  T_285751980_132000_Estación_Transformadora_Luján/RConn2 -- L_285751980/LConn2
  L_285751980/LConn3 -- T_285751980_132000_Estación_Transformadora_Luján/RConn3 -- bus233/LConn1
  T_323007027__/RConn1 -- L_323007027/LConn1
  T_323007027__/RConn2 -- L_323007027/LConn2
  L_323007027/LConn3 -- T_323007027__/RConn3 -- bus234/LConn1
  T_163331032__/RConn1 -- L_163331032/LConn1
  T_163331032__/RConn2 -- L_163331032/LConn2
  L_163331032/LConn3 -- T_163331032__/RConn3 -- bus235/LConn1
  T_323007032__/RConn1 -- L_323007032/LConn1
  T_323007032__/RConn2 -- L_323007032/LConn2
  L_323007032/LConn3 -- T_323007032__/RConn3 -- bus236/LConn1
  T_323007054__/RConn1 -- L_323007054/LConn1
  T_323007054__/RConn2 -- L_323007054/LConn2
  L_323007054/LConn3 -- T_323007054__/RConn3 -- bus237/LConn1
  T_413160973__/RConn1 -- L_413160973/LConn1
  T_413160973__/RConn2 -- L_413160973/LConn2
  L_413160973/LConn3 -- T_413160973__/RConn3 -- bus238/LConn1
  T_413160958__/RConn1 -- L_413160958/LConn1
  T_413160958__/RConn2 -- L_413160958/LConn2
  L_413160958/LConn3 -- T_413160958__/RConn3 -- bus239/LConn1
  T_323007058__/RConn1 -- L_323007058/LConn1
  T_323007058__/RConn2 -- L_323007058/LConn2
  L_323007058/LConn3 -- T_323007058__/RConn3 -- bus240/LConn1
  T_321536940__/RConn1 -- L_321536940/LConn1
  T_321536940__/RConn2 -- L_321536940/LConn2
  L_321536940/LConn3 -- T_321536940__/RConn3 -- bus241/LConn1
  T_322915916__/RConn1 -- L_322915916/LConn1
  T_322915916__/RConn2 -- L_322915916/LConn2
  L_322915916/LConn3 -- T_322915916__/RConn3 -- bus242/LConn1
  T_255783500__/RConn1 -- L_255783500/LConn1
  T_255783500__/RConn2 -- L_255783500/LConn2
  L_255783500/LConn3 -- T_255783500__/RConn3 -- bus243/LConn1
  T_277739294__/RConn1 -- L_277739294/LConn1
  T_277739294__/RConn2 -- L_277739294/LConn2
  L_277739294/LConn3 -- T_277739294__/RConn3 -- bus244/LConn1
  T_314623617__/RConn1 -- L_314623617/LConn1
  T_314623617__/RConn2 -- L_314623617/LConn2
  L_314623617/LConn3 -- T_314623617__/RConn3 -- bus245/LConn1
  T_348409732__/RConn1 -- L_348409732/LConn1
  T_348409732__/RConn2 -- L_348409732/LConn2
  L_348409732/LConn3 -- T_348409732__/RConn3 -- bus246/LConn1
  T_323007050__/RConn1 -- L_323007050/LConn1
  T_323007050__/RConn2 -- L_323007050/LConn2
  L_323007050/LConn3 -- T_323007050__/RConn3 -- bus247/LConn1
  T_204494929__Estação_Conversora_de_Frequencia_de_Uruguaiana/RConn1 -- L_204494929/LConn1
  T_204494929__Estação_Conversora_de_Frequencia_de_Uruguaiana/RConn2 -- L_204494929/LConn2
  L_204494929/LConn3 -- T_204494929__Estação_Conversora_de_Frequencia_de_Uruguaiana/RConn3 -- bus248/LConn1
  T_204494933__/RConn1 -- L_204494933/LConn1
  T_204494933__/RConn2 -- L_204494933/LConn2
  L_204494933/LConn3 -- T_204494933__/RConn3 -- bus249/LConn1
  T_248861779__/RConn1 -- L_248861779/LConn1
  T_248861779__/RConn2 -- L_248861779/LConn2
  L_248861779/LConn3 -- T_248861779__/RConn3 -- bus250/LConn1
  T_323105942__/RConn1 -- L_323105942/LConn1
  T_323105942__/RConn2 -- L_323105942/LConn2
  L_323105942/LConn3 -- T_323105942__/RConn3 -- bus251/LConn1
  T_145419356__/RConn1 -- L_145419356/LConn1
  T_145419356__/RConn2 -- L_145419356/LConn2
  L_145419356/LConn3 -- T_145419356__/RConn3 -- bus252/LConn1
  T_422118006__/RConn1 -- L_422118006/LConn1
  T_422118006__/RConn2 -- L_422118006/LConn2
  L_422118006/LConn3 -- T_422118006__/RConn3 -- bus253/LConn1
  T_130194705__/RConn1 -- L_130194705/LConn1
  T_130194705__/RConn2 -- L_130194705/LConn2
  L_130194705/LConn3 -- T_130194705__/RConn3 -- bus254/LConn1
  T_284287249__Subestación_Sobral/RConn1 -- L_284287249/LConn1
  T_284287249__Subestación_Sobral/RConn2 -- L_284287249/LConn2
  L_284287249/LConn3 -- T_284287249__Subestación_Sobral/RConn3 -- bus255/LConn1
  T_277938914__/RConn1 -- L_277938914/LConn1
  T_277938914__/RConn2 -- L_277938914/LConn2
  L_277938914/LConn3 -- T_277938914__/RConn3 -- bus256/LConn1
  T_309033575__/RConn1 -- L_309033575/LConn1
  T_309033575__/RConn2 -- L_309033575/LConn2
  L_309033575/LConn3 -- T_309033575__/RConn3 -- bus257/LConn1
  T_251093639_132000_Estación_Transformadora_Verónica/RConn1 -- L_251093639/LConn1
  T_251093639_132000_Estación_Transformadora_Verónica/RConn2 -- L_251093639/LConn2
  L_251093639/LConn3 -- T_251093639_132000_Estación_Transformadora_Verónica/RConn3 -- bus258/LConn1
  T_299924594__Estación_Pico_Truncado_I/RConn1 -- L_299924594/LConn1
  T_299924594__Estación_Pico_Truncado_I/RConn2 -- L_299924594/LConn2
  L_299924594/LConn3 -- T_299924594__Estación_Pico_Truncado_I/RConn3 -- bus259/LConn1
  T_223678069__Estación_transformadora_Puerto_Deseado/RConn1 -- L_223678069/LConn1
  T_223678069__Estación_transformadora_Puerto_Deseado/RConn2 -- L_223678069/LConn2
  L_223678069/LConn3 -- T_223678069__Estación_transformadora_Puerto_Deseado/RConn3 -- bus260/LConn1
  T_299598854__Estación_transformadora_Las_Heras/RConn1 -- L_299598854/LConn1
  T_299598854__Estación_transformadora_Las_Heras/RConn2 -- L_299598854/LConn2
  L_299598854/LConn3 -- T_299598854__Estación_transformadora_Las_Heras/RConn3 -- bus261/LConn1
  T_129988212__Subestación_Transformadora_Transba/RConn1 -- L_129988212/LConn1
  T_129988212__Subestación_Transformadora_Transba/RConn2 -- L_129988212/LConn2
  L_129988212/LConn3 -- T_129988212__Subestación_Transformadora_Transba/RConn3 -- bus262/LConn1
  T_322781304__/RConn1 -- L_322781304/LConn1
  T_322781304__/RConn2 -- L_322781304/LConn2
  L_322781304/LConn3 -- T_322781304__/RConn3 -- bus263/LConn1
  T_208425737__Eléctrica/RConn1 -- L_208425737/LConn1
  T_208425737__Eléctrica/RConn2 -- L_208425737/LConn2
  L_208425737/LConn3 -- T_208425737__Eléctrica/RConn3 -- bus264/LConn1
  T_210279051__Estación_Transformadora/RConn1 -- L_210279051/LConn1
  T_210279051__Estación_Transformadora/RConn2 -- L_210279051/LConn2
  L_210279051/LConn3 -- T_210279051__Estación_Transformadora/RConn3 -- bus265/LConn1
  T_283604831__/RConn1 -- L_283604831/LConn1
  T_283604831__/RConn2 -- L_283604831/LConn2
  L_283604831/LConn3 -- T_283604831__/RConn3 -- bus266/LConn1
  T_310571477__/RConn1 -- L_310571477/LConn1
  T_310571477__/RConn2 -- L_310571477/LConn2
  L_310571477/LConn3 -- T_310571477__/RConn3 -- bus267/LConn1
  T_286336657__/RConn1 -- L_286336657/LConn1
  T_286336657__/RConn2 -- L_286336657/LConn2
  L_286336657/LConn3 -- T_286336657__/RConn3 -- bus268/LConn1
  T_413160959__/RConn1 -- L_413160959/LConn1
  T_413160959__/RConn2 -- L_413160959/LConn2
  L_413160959/LConn3 -- T_413160959__/RConn3 -- bus269/LConn1
  T_196031429__/RConn1 -- L_196031429/LConn1
  T_196031429__/RConn2 -- L_196031429/LConn2
  L_196031429/LConn3 -- T_196031429__/RConn3 -- bus270/LConn1
  T_353728814__Estaciòn_Transformadora_San_Miguel/RConn1 -- L_353728814/LConn1
  T_353728814__Estaciòn_Transformadora_San_Miguel/RConn2 -- L_353728814/LConn2
  L_353728814/LConn3 -- T_353728814__Estaciòn_Transformadora_San_Miguel/RConn3 -- bus271/LConn1
  T_290602502__/RConn1 -- L_290602502/LConn1
  T_290602502__/RConn2 -- L_290602502/LConn2
  L_290602502/LConn3 -- T_290602502__/RConn3 -- bus272/LConn1
  T_432044715__/RConn1 -- L_432044715/LConn1
  T_432044715__/RConn2 -- L_432044715/LConn2
  L_432044715/LConn3 -- T_432044715__/RConn3 -- bus273/LConn1
  T_431976152__/RConn1 -- L_431976152/LConn1
  T_431976152__/RConn2 -- L_431976152/LConn2
  L_431976152/LConn3 -- T_431976152__/RConn3 -- bus274/LConn1
  T_306029239__/RConn1 -- L_306029239/LConn1
  T_306029239__/RConn2 -- L_306029239/LConn2
  L_306029239/LConn3 -- T_306029239__/RConn3 -- bus275/LConn1
  T_329781271__/RConn1 -- L_329781271/LConn1
  T_329781271__/RConn2 -- L_329781271/LConn2
  L_329781271/LConn3 -- T_329781271__/RConn3 -- bus276/LConn1
  T_429251282_132000_Estación_Rawson/RConn1 -- L_429251282/LConn1
  T_429251282_132000_Estación_Rawson/RConn2 -- L_429251282/LConn2
  L_429251282/LConn3 -- T_429251282_132000_Estación_Rawson/RConn3 -- bus277/LConn1
  T_429251283_132000_Estación_Trelew/RConn1 -- L_429251283/LConn1
  T_429251283_132000_Estación_Trelew/RConn2 -- L_429251283/LConn2
  L_429251283/LConn3 -- T_429251283_132000_Estación_Trelew/RConn3 -- bus278/LConn1
  T_429251281_132000_Estación_Parque_eólico_Rawson/RConn1 -- L_429251281/LConn1
  T_429251281_132000_Estación_Parque_eólico_Rawson/RConn2 -- L_429251281/LConn2
  L_429251281/LConn3 -- T_429251281_132000_Estación_Parque_eólico_Rawson/RConn3 -- bus279/LConn1
  T_317981558__Subestación_transformadora_Los_Perales_2/RConn1 -- L_317981558/LConn1
  T_317981558__Subestación_transformadora_Los_Perales_2/RConn2 -- L_317981558/LConn2
  L_317981558/LConn3 -- T_317981558__Subestación_transformadora_Los_Perales_2/RConn3 -- bus280/LConn1
  T_277938913__/RConn1 -- L_277938913/LConn1
  T_277938913__/RConn2 -- L_277938913/LConn2
  L_277938913/LConn3 -- T_277938913__/RConn3 -- bus281/LConn1
  T_277938915__/RConn1 -- L_277938915/LConn1
  T_277938915__/RConn2 -- L_277938915/LConn2
  L_277938915/LConn3 -- T_277938915__/RConn3 -- bus282/LConn1
  T_321354632__/RConn1 -- L_321354632/LConn1
  T_321354632__/RConn2 -- L_321354632/LConn2
  L_321354632/LConn3 -- T_321354632__/RConn3 -- bus283/LConn1
  T_328056071__/RConn1 -- L_328056071/LConn1
  T_328056071__/RConn2 -- L_328056071/LConn2
  L_328056071/LConn3 -- T_328056071__/RConn3 -- bus284/LConn1
  T_363050268__Estacion_Transformadora_Villa_Mercedes/RConn1 -- L_363050268/LConn1
  T_363050268__Estacion_Transformadora_Villa_Mercedes/RConn2 -- L_363050268/LConn2
  L_363050268/LConn3 -- T_363050268__Estacion_Transformadora_Villa_Mercedes/RConn3 -- bus285/LConn1
  T_248651545__/RConn1 -- L_248651545/LConn1
  T_248651545__/RConn2 -- L_248651545/LConn2
  L_248651545/LConn3 -- T_248651545__/RConn3 -- bus286/LConn1
  T_22984932__Subestación_de_EDELAP/RConn1 -- L_22984932/LConn1
  T_22984932__Subestación_de_EDELAP/RConn2 -- L_22984932/LConn2
  L_22984932/LConn3 -- T_22984932__Subestación_de_EDELAP/RConn3 -- bus287/LConn1
  T_431767371__/RConn1 -- L_431767371/LConn1
  T_431767371__/RConn2 -- L_431767371/LConn2
  L_431767371/LConn3 -- T_431767371__/RConn3 -- bus288/LConn1
  T_241864152__/RConn1 -- L_241864152/LConn1
  T_241864152__/RConn2 -- L_241864152/LConn2
  L_241864152/LConn3 -- T_241864152__/RConn3 -- bus289/LConn1
  T_154839518__TRANSBA___Subestación_Olavarría___132kV/RConn1 -- L_154839518/LConn1
  T_154839518__TRANSBA___Subestación_Olavarría___132kV/RConn2 -- L_154839518/LConn2
  L_154839518/LConn3 -- T_154839518__TRANSBA___Subestación_Olavarría___132kV/RConn3 -- bus290/LConn1
  T_211179868__/RConn1 -- L_211179868/LConn1
  T_211179868__/RConn2 -- L_211179868/LConn2
  L_211179868/LConn3 -- T_211179868__/RConn3 -- bus291/LConn1
  T_277739297__/RConn1 -- L_277739297/LConn1
  T_277739297__/RConn2 -- L_277739297/LConn2
  L_277739297/LConn3 -- T_277739297__/RConn3 -- bus292/LConn1
  T_277739295_132000_/RConn1 -- L_277739295/LConn1
  T_277739295_132000_/RConn2 -- L_277739295/LConn2
  L_277739295/LConn3 -- T_277739295_132000_/RConn3 -- bus293/LConn1
  T_277739298__/RConn1 -- L_277739298/LConn1
  T_277739298__/RConn2 -- L_277739298/LConn2
  L_277739298/LConn3 -- T_277739298__/RConn3 -- bus294/LConn1
  T_321354631__/RConn1 -- L_321354631/LConn1
  T_321354631__/RConn2 -- L_321354631/LConn2
  L_321354631/LConn3 -- T_321354631__/RConn3 -- bus295/LConn1
  T_340060050_500000_Estación_Transformadora_Centro/RConn1 -- L_340060050/LConn1
  T_340060050_500000_Estación_Transformadora_Centro/RConn2 -- L_340060050/LConn2
  L_340060050/LConn3 -- T_340060050_500000_Estación_Transformadora_Centro/RConn3 -- bus296/LConn1
  T_97399680_500000_Estación_Transformadora_San_Isidro/RConn1 -- L_97399680/LConn1
  T_97399680_500000_Estación_Transformadora_San_Isidro/RConn2 -- L_97399680/LConn2
  L_97399680/LConn3 -- T_97399680_500000_Estación_Transformadora_San_Isidro/RConn3 -- bus297/LConn1
  T_392660851__/RConn1 -- L_392660851/LConn1
  T_392660851__/RConn2 -- L_392660851/LConn2
  L_392660851/LConn3 -- T_392660851__/RConn3 -- bus298/LConn1
  T_326097046__/RConn1 -- L_326097046/LConn1
  T_326097046__/RConn2 -- L_326097046/LConn2
  L_326097046/LConn3 -- T_326097046__/RConn3 -- bus299/LConn1
  T_230329765__/RConn1 -- L_230329765/LConn1
  T_230329765__/RConn2 -- L_230329765/LConn2
  L_230329765/LConn3 -- T_230329765__/RConn3 -- bus300/LConn1
  T_322781303__/RConn1 -- L_322781303/LConn1
  T_322781303__/RConn2 -- L_322781303/LConn2
  L_322781303/LConn3 -- T_322781303__/RConn3 -- bus301/LConn1
  T_321398721__/RConn1 -- L_321398721/LConn1
  T_321398721__/RConn2 -- L_321398721/LConn2
  L_321398721/LConn3 -- T_321398721__/RConn3 -- bus302/LConn1
  T_259688907__/RConn1 -- L_259688907/LConn1
  T_259688907__/RConn2 -- L_259688907/LConn2
  L_259688907/LConn3 -- T_259688907__/RConn3 -- bus303/LConn1
  T_431598950__/RConn1 -- L_431598950/LConn1
  T_431598950__/RConn2 -- L_431598950/LConn2
  L_431598950/LConn3 -- T_431598950__/RConn3 -- bus304/LConn1
  T_164577670__Estación_Electrica/RConn1 -- L_164577670/LConn1
  T_164577670__Estación_Electrica/RConn2 -- L_164577670/LConn2
  L_164577670/LConn3 -- T_164577670__Estación_Electrica/RConn3 -- bus305/LConn1
  T_164673290__/RConn1 -- L_164673290/LConn1
  T_164673290__/RConn2 -- L_164673290/LConn2
  L_164673290/LConn3 -- T_164673290__/RConn3 -- bus306/LConn1
  T_273522974__/RConn1 -- L_273522974/LConn1
  T_273522974__/RConn2 -- L_273522974/LConn2
  L_273522974/LConn3 -- T_273522974__/RConn3 -- bus307/LConn1
  T_285554517__/RConn1 -- L_285554517/LConn1
  T_285554517__/RConn2 -- L_285554517/LConn2
  L_285554517/LConn3 -- T_285554517__/RConn3 -- bus308/LConn1
  T_172440613__/RConn1 -- L_172440613/LConn1
  T_172440613__/RConn2 -- L_172440613/LConn2
  L_172440613/LConn3 -- T_172440613__/RConn3 -- bus309/LConn1
  T_193242927__/RConn1 -- L_193242927/LConn1
  T_193242927__/RConn2 -- L_193242927/LConn2
  L_193242927/LConn3 -- T_193242927__/RConn3 -- bus310/LConn1
  T_178248568__/RConn1 -- L_178248568/LConn1
  T_178248568__/RConn2 -- L_178248568/LConn2
  L_178248568/LConn3 -- T_178248568__/RConn3 -- bus311/LConn1
  T_242365381__/RConn1 -- L_242365381/LConn1
  T_242365381__/RConn2 -- L_242365381/LConn2
  L_242365381/LConn3 -- T_242365381__/RConn3 -- bus312/LConn1
  T_277132135_220000_Estación_transformadora_Villa_Lía/RConn1 -- L_277132135/LConn1
  T_277132135_220000_Estación_transformadora_Villa_Lía/RConn2 -- L_277132135/LConn2
  L_277132135/LConn3 -- T_277132135_220000_Estación_transformadora_Villa_Lía/RConn3 -- bus313/LConn1
  T_310114524__Subestación_Edenor/RConn1 -- L_310114524/LConn1
  T_310114524__Subestación_Edenor/RConn2 -- L_310114524/LConn2
  L_310114524/LConn3 -- T_310114524__Subestación_Edenor/RConn3 -- bus314/LConn1
  T_188360578__/RConn1 -- L_188360578/LConn1
  T_188360578__/RConn2 -- L_188360578/LConn2
  L_188360578/LConn3 -- T_188360578__/RConn3 -- bus315/LConn1
  T_247830316__/RConn1 -- L_247830316/LConn1
  T_247830316__/RConn2 -- L_247830316/LConn2
  L_247830316/LConn3 -- T_247830316__/RConn3 -- bus316/LConn1
  T_413038969__/RConn1 -- L_413038969/LConn1
  T_413038969__/RConn2 -- L_413038969/LConn2
  L_413038969/LConn3 -- T_413038969__/RConn3 -- bus317/LConn1
  T_277426564__/RConn1 -- L_277426564/LConn1
  T_277426564__/RConn2 -- L_277426564/LConn2
  L_277426564/LConn3 -- T_277426564__/RConn3 -- bus318/LConn1
  T_176046623__/RConn1 -- L_176046623/LConn1
  T_176046623__/RConn2 -- L_176046623/LConn2
  L_176046623/LConn3 -- T_176046623__/RConn3 -- bus319/LConn1
  T_218457595__/RConn1 -- L_218457595/LConn1
  T_218457595__/RConn2 -- L_218457595/LConn2
  L_218457595/LConn3 -- T_218457595__/RConn3 -- bus320/LConn1
  T_110339851__Estación_Transformadora_Puerto_Bastiani/RConn1 -- L_110339851/LConn1
  T_110339851__Estación_Transformadora_Puerto_Bastiani/RConn2 -- L_110339851/LConn2
  L_110339851/LConn3 -- T_110339851__Estación_Transformadora_Puerto_Bastiani/RConn3 -- bus321/LConn1
  T_258696364__/RConn1 -- L_258696364/LConn1
  T_258696364__/RConn2 -- L_258696364/LConn2
  L_258696364/LConn3 -- T_258696364__/RConn3 -- bus322/LConn1
  T_258696366__/RConn1 -- L_258696366/LConn1
  T_258696366__/RConn2 -- L_258696366/LConn2
  L_258696366/LConn3 -- T_258696366__/RConn3 -- bus323/LConn1
  T_305162903__/RConn1 -- L_305162903/LConn1
  T_305162903__/RConn2 -- L_305162903/LConn2
  L_305162903/LConn3 -- T_305162903__/RConn3 -- bus324/LConn1
  T_203954946_500000_Estación_transformadora_Colonia_Elía/RConn1 -- L_203954946/LConn1
  T_203954946_500000_Estación_transformadora_Colonia_Elía/RConn2 -- L_203954946/LConn2
  L_203954946/LConn3 -- T_203954946_500000_Estación_transformadora_Colonia_Elía/RConn3 -- bus325/LConn1
  T_190845501__/RConn1 -- L_190845501/LConn1
  T_190845501__/RConn2 -- L_190845501/LConn2
  L_190845501/LConn3 -- T_190845501__/RConn3 -- bus326/LConn1
  T_274067533__/RConn1 -- L_274067533/LConn1
  T_274067533__/RConn2 -- L_274067533/LConn2
  L_274067533/LConn3 -- T_274067533__/RConn3 -- bus327/LConn1
  T_186421221__/RConn1 -- L_186421221/LConn1
  T_186421221__/RConn2 -- L_186421221/LConn2
  L_186421221/LConn3 -- T_186421221__/RConn3 -- bus328/LConn1
  T_247820688__/RConn1 -- L_247820688/LConn1
  T_247820688__/RConn2 -- L_247820688/LConn2
  L_247820688/LConn3 -- T_247820688__/RConn3 -- bus329/LConn1
  T_89373622__/RConn1 -- L_89373622/LConn1
  T_89373622__/RConn2 -- L_89373622/LConn2
  L_89373622/LConn3 -- T_89373622__/RConn3 -- bus330/LConn1
  T_247830317__/RConn1 -- L_247830317/LConn1
  T_247830317__/RConn2 -- L_247830317/LConn2
  L_247830317/LConn3 -- T_247830317__/RConn3 -- bus331/LConn1
  T_213568638__/RConn1 -- L_213568638/LConn1
  T_213568638__/RConn2 -- L_213568638/LConn2
  L_213568638/LConn3 -- T_213568638__/RConn3 -- bus332/LConn1
  T_71775909__Central_Termoeléctrica_Piedra_Buena/RConn1 -- L_71775909/LConn1
  T_71775909__Central_Termoeléctrica_Piedra_Buena/RConn2 -- L_71775909/LConn2
  L_71775909/LConn3 -- T_71775909__Central_Termoeléctrica_Piedra_Buena/RConn3 -- bus333/LConn1
  T_305027751__/RConn1 -- L_305027751/LConn1
  T_305027751__/RConn2 -- L_305027751/LConn2
  L_305027751/LConn3 -- T_305027751__/RConn3 -- bus334/LConn1
  T_215284908_500000_Estación_Transformadora_Manuel_Belgrano/RConn1 -- L_215284908/LConn1
  T_215284908_500000_Estación_Transformadora_Manuel_Belgrano/RConn2 -- L_215284908/LConn2
  L_215284908/LConn3 -- T_215284908_500000_Estación_Transformadora_Manuel_Belgrano/RConn3 -- bus335/LConn1
  T_213578175__Subestación_eléctrica/RConn1 -- L_213578175/LConn1
  T_213578175__Subestación_eléctrica/RConn2 -- L_213578175/LConn2
  L_213578175/LConn3 -- T_213578175__Subestación_eléctrica/RConn3 -- bus336/LConn1
  T_253226994__/RConn1 -- L_253226994/LConn1
  T_253226994__/RConn2 -- L_253226994/LConn2
  L_253226994/LConn3 -- T_253226994__/RConn3 -- bus337/LConn1
  T_314753857__Estación_transformadora_Piedrabuena/RConn1 -- L_314753857/LConn1
  T_314753857__Estación_transformadora_Piedrabuena/RConn2 -- L_314753857/LConn2
  L_314753857/LConn3 -- T_314753857__Estación_transformadora_Piedrabuena/RConn3 -- bus338/LConn1
  T_303134158__/RConn1 -- L_303134158/LConn1
  T_303134158__/RConn2 -- L_303134158/LConn2
  L_303134158/LConn3 -- T_303134158__/RConn3 -- bus339/LConn1
  T_173947403__Transener_S_A_/RConn1 -- L_173947403/LConn1
  T_173947403__Transener_S_A_/RConn2 -- L_173947403/LConn2
  L_173947403/LConn3 -- T_173947403__Transener_S_A_/RConn3 -- bus340/LConn1
  T_306717418__/RConn1 -- L_306717418/LConn1
  T_306717418__/RConn2 -- L_306717418/LConn2
  L_306717418/LConn3 -- T_306717418__/RConn3 -- bus341/LConn1
  T_213192902__/RConn1 -- L_213192902/LConn1
  T_213192902__/RConn2 -- L_213192902/LConn2
  L_213192902/LConn3 -- T_213192902__/RConn3 -- bus342/LConn1
  T_213192904__/RConn1 -- L_213192904/LConn1
  T_213192904__/RConn2 -- L_213192904/LConn2
  L_213192904/LConn3 -- T_213192904__/RConn3 -- bus343/LConn1
  T_213192903__/RConn1 -- L_213192903/LConn1
  T_213192903__/RConn2 -- L_213192903/LConn2
  L_213192903/LConn3 -- T_213192903__/RConn3 -- bus344/LConn1
  T_26119134__Transener_S_A_/RConn1 -- L_26119134/LConn1
  T_26119134__Transener_S_A_/RConn2 -- L_26119134/LConn2
  L_26119134/LConn3 -- T_26119134__Transener_S_A_/RConn3 -- bus345/LConn1
  T_221357412__Central_Hidroeléctrica_de_Yacyretá_Apipé/RConn1 -- L_221357412/LConn1
  T_221357412__Central_Hidroeléctrica_de_Yacyretá_Apipé/RConn2 -- L_221357412/LConn2
  L_221357412/LConn3 -- T_221357412__Central_Hidroeléctrica_de_Yacyretá_Apipé/RConn3 -- bus346/LConn1
  T_323007074__/RConn1 -- L_323007074/LConn1
  T_323007074__/RConn2 -- L_323007074/LConn2
  L_323007074/LConn3 -- T_323007074__/RConn3 -- bus347/LConn1
  T_305103439__/RConn1 -- L_305103439/LConn1
  T_305103439__/RConn2 -- L_305103439/LConn2
  L_305103439/LConn3 -- T_305103439__/RConn3 -- bus348/LConn1
  T_305103437__/RConn1 -- L_305103437/LConn1
  T_305103437__/RConn2 -- L_305103437/LConn2
  L_305103437/LConn3 -- T_305103437__/RConn3 -- bus349/LConn1
  T_204484095__/RConn1 -- L_204484095/LConn1
  T_204484095__/RConn2 -- L_204484095/LConn2
  L_204484095/LConn3 -- T_204484095__/RConn3 -- bus350/LConn1
